simulink model "Copy_of_ENV"  (R2024b)
settings: Solver=FixedStepAuto  StartTime=0.0  StopTime=10.0  RelTol=1e-3  EnableMultiTasking=on
libraries: stm32blockslib x27, canmsglib x9, stm32f4xxblockslib x6, simulink x5
(part 1 of 2)
settings Model: DataDictionary=Master_Dictionary.sldd  STM32="{\"DigitalPortRead\":[{\"ID\":\"ENV:103\"},{\"ID\":\"ENV:734\"}],\"DigitalPortWrite\":[{\"ID\":\"ENV:105\"},{\"ID\":\"ENV:104\"},{\"ID\":\"ENV:735\"},{\"ID\":\"ENV:739\"}],\"SPIControllerTransfer\":[{\"ID\":\"ENV:28\"},{\"ID\":\"ENV:29\"},{\"ID\":\"ENV:30\"},{\"ID\":\"ENV:31\"},{\"ID\":\"ENV:32\"},{\"ID\":\"ENV:33\"},{\"ID\":\"ENV:89\"},{\"ID\":\"ENV:90\"},{\"ID\":\"ENV:91\"},{\"ID\":\"ENV:92\"},{\"ID\":\"ENV:661\"},{\"ID\":\"ENV:662\"},{\"ID\":\"ENV:663\"},{\"ID\":\"ENV:664\"},{\"ID\":\"ENV:665\"},{\"ID\":\"ENV:666\"},{\"ID\":\"ENV:667\"},{\"ID\":\"ENV:668\"},{\"ID\":\"ENV:697\"},{\"ID\":\"ENV:785\"},{\"ID\":\"ENV:784\"},{\"ID\":\"ENV:783\"},{\"ID\":\"ENV:782\"},{\"ID\":\"ENV:781\"},{\"ID\":\"ENV:780\"},{\"ID\":\"ENV:779\"},{\"ID\":\"ENV:778\"}]}"  Creator=Will  LastModifiedBy=Will
settings OptimizationCC: DefaultParameterBehavior=Inlined  EnhancedBackFolding=on  PassReuseOutputArgsAs=Individual arguments  ZeroExternalMemoryAtStartup=off  ZeroInternalMemoryAtStartup=off  MaxStackSize=8192  OptimizeBlockOrder=speed  DifferentSizesBufferReuse=on  OptimizationCustomize=off  EfficientTunableParamExpr=on
settings DebuggingCC: ParameterTunabilityLossMsg=error
settings HardwareCC: ProdBitPerPointer=32  ProdBitPerSizeT=32  ProdBitPerPtrDiffT=32  ProdLargestAtomicInteger=Long  ProdLargestAtomicFloat=Double  ProdWordSize=32  ProdLongLongMode=on  ProdHWDeviceType=ARM Compatible->ARM Cortex-M
settings SFSimCC: MATLABDynamicMemAlloc=off
settings RTWCC: Description=Embedded Coder  SystemTargetFile=ert.tlc  HardwareBoard=STM32H7xx Based (Single-core)  TemplateMakefile=ert_default_tmf  Toolchain=GNU Tools for ARM Embedded Processors
settings CodeAppCC: ForceParamTrailComments=on  IgnoreCustomStorageClasses=off  OperatorAnnotations=on  SimulinkDataObjDesc=on  SFDataObjDesc=on  InsertBlockDesc=on
settings ERTTargetCC: TargetLangStandard=C99 (ISO)  CodeReplacementLibrary=ARM Cortex-M  ExtModeTransport=3  ExtModeStaticAlloc=on  ExtModeStaticAllocSize=2048  ExtModeMexFile=ext_xcp  ExtModeIntrfLevel=Level2 - Open

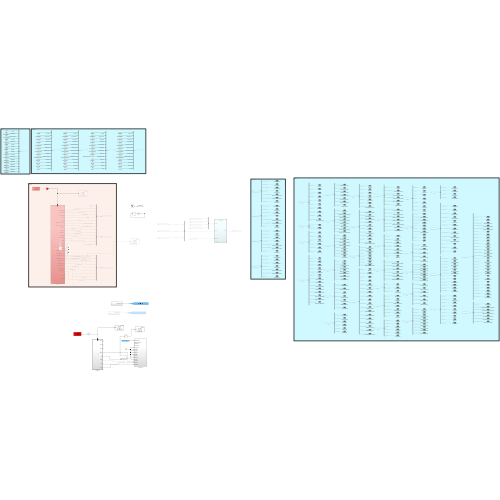
[thumbnail: Simulink's stored preview of the top-level diagram]
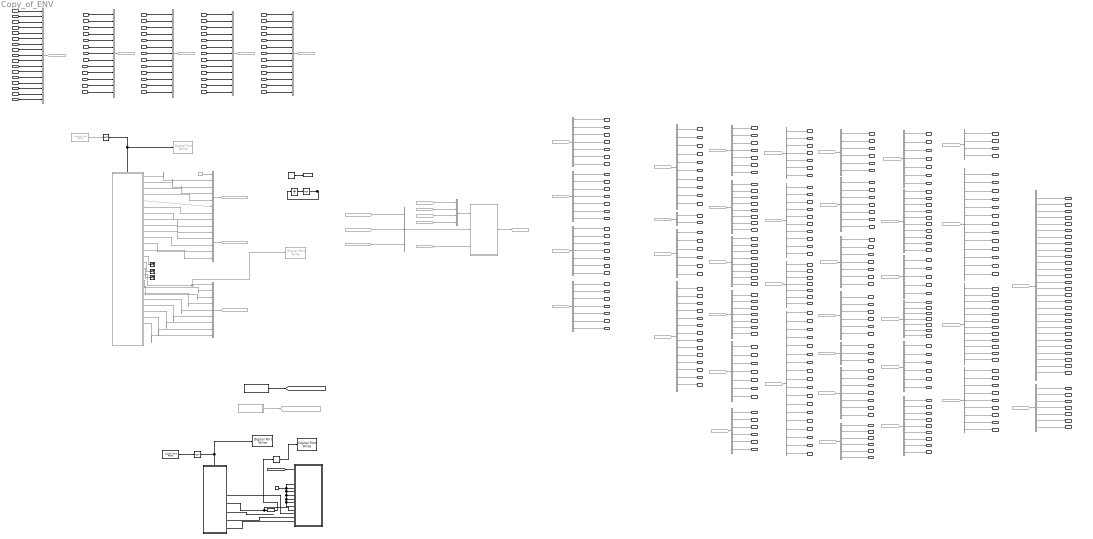
== system Copy_of_ENV ==
  note: CAN3
  note: CAN3
  note: CAN 1&2
  note: CAN1&2
  note: CAN4
  nMotorRL : Inport
  BInvDCOnRLIn : Inport  Port=2
  BInvErrorRL : Inport  Port=3
  BInvOnRLIn : Inport  Port=4
  BInvQuitDcOnRL : Inport  Port=5
  BQuitInvOnRL : Inport  Port=6
  BInvSysReadyRL : Inport  Port=7
  BInvWarnRL : Inport  Port=8
  MMotorMeasuredRL : Inport  Port=9
  NInvDTCRL : Inport  Port=10
  TMotorRL : Inport  Port=11
  VDCInvRL : Inport  Port=12
  TInvRL : Inport  Port=13
  nMotorRR : Inport  Port=14
  BInvDCOnRRIn : Inport  Port=15
  BInvErrorRR : Inport  Port=16
  BInvOnRRIn : Inport  Port=17
  BInvQuitDcOnRR : Inport  Port=18
  BQuitInvOnRR : Inport  Port=19
  BInvSysReadyRR : Inport  Port=20
  BInvWarnRR : Inport  Port=21
  MMotorMeasuredRR : Inport  Port=22
  NInvDTCRR : Inport  Port=23
  TMotorRR : Inport  Port=24
  VDCInvRR : Inport  Port=25
  TInvRR : Inport  Port=26
  nMotorFL : Inport  Port=27
  BInvDCOnFLIn : Inport  Port=28
  BInvErrorFL : Inport  Port=29
  BInvOnFLIn : Inport  Port=30
  BInvQuitDcOnFL : Inport  Port=31
  BQuitInvOnFL : Inport  Port=32
  BInvSysReadyFL : Inport  Port=33
  BInvWarnFL : Inport  Port=34
  MMotorMeasuredFL : Inport  Port=35
  NInvDTCFL : Inport  Port=36
  TMotorFL : Inport  Port=37
  VDCInvFL : Inport  Port=38
  TInvFL : Inport  Port=39
  nMotorFR : Inport  Port=40
  BInvDCOnFRIn : Inport  Port=41
  BInvErrorFR : Inport  Port=42
  BInvOnFRIn : Inport  Port=43
  BInvQuitDcOnFR : Inport  Port=44
  BQuitInvOnFR : Inport  Port=45
  BInvSysReadyFR : Inport  Port=46
  BInvWarnFR : Inport  Port=47
  MMotorMeasuredFR : Inport  Port=48
  NInvDTCFR : Inport  Port=49
  TMotorFR : Inport  Port=50
  VDCInvFR : Inport  Port=51
  TInvFR : Inport  Port=52
  IIVTS : Inport  Port=53
  IBMSHallEffect : Inport  Port=54
  VDCAccumulator : Inport  Port=55
  TCellMin : Inport  Port=56
  VCellAverage : Inport  Port=57
  VCellMax : Inport  Port=58
  TCellMax : Inport  Port=59
  IBMSDCL : Inport  Port=60
  VCellMin : Inport  Port=61
  RCellAverage : Inport  Port=62
  BBalancingOn : Inport  Port=63
  BBMSP0A0C : Inport  Port=64  OutDataTypeStr=boolean
  BBMSP0A0E : Inport  Port=65
  BBMSP0A10 : Inport  Port=66
  BBMSP0A80 : Inport  Port=67
  BBMSP0AC0 : Inport  Port=68
  BBMSP0AFA : Inport  Port=69
  0x1A0 : From  Commented=on  GotoTag=Global
  0x1A1 : From  Commented=on  GotoTag=Global
  0x1A2 : From  Commented=on  GotoTag=Global
  0x{202..203,205..207,210..217,220..223,250..254,300..302,603,700..703} (30 alike) : From  Commented=on  GotoTag=Global
  Bus Creator : BusCreator  Commented=on  Inputs=3  OutDataTypeStr=Bus: CAN3Bus
  Bus Creator14 : BusCreator  Commented=on  Inputs=13  OutDataTypeStr=Bus: InverterFL
  Bus Creator15 : BusCreator  Commented=on  Inputs=13  OutDataTypeStr=Bus: InverterFR
  Bus Creator17 : BusCreator  Commented=on  Inputs=13  OutDataTypeStr=Bus: InverterRL
  Bus Creator18 : BusCreator  Commented=on  Inputs=17  OutDataTypeStr=Bus: BMS
  Bus Creator19 : BusCreator  Commented=on  Inputs=13  OutDataTypeStr=Bus: InverterRR
  Bus Creator2 : BusCreator  Commented=on  Inputs=8  OutDataTypeStr=Bus: DDU7
  Bus Creator3 : BusCreator  Commented=on  Inputs=6  OutDataTypeStr=Bus: IMU
      settings: InheritFromInputs=off
  Bus Creator4 : BusCreator  Commented=on  Inputs=9  OutDataTypeStr=Bus: STW
  Bus Selector : BusSelector  Commented=on  OutputSignals=TorqueControl.MFLFinal,TorqueControl.MFRFinal,TorqueControl.MRLFinal,TorqueControl.MRRFinal,BMSSignals.IIVTS,Systems.PActual,Systems.BBrakeError,Systems.BThrottleError,Systems.BOverpower,Limitations.BDischargeAllowed
  Bus Selector1 : BusSelector  Commented=on  OutputSignals=Systems.vChassis,Systems.PEnergyMeter
  Bus Selector10 : BusSelector  Commented=on  OutputSignals=TorqueControl.MTotalRequested,TorqueControl.rSlipRatioOptimal,TorqueControl.aCamberFL,TorqueControl.aCamberFR,TorqueControl.aCamberRL,TorqueControl.aCamberRR,TorqueControl.FTotalLateralLoadTransfer
  Bus Selector11 : BusSelector  Commented=on  OutputSignals=Systems.BTVOnEM,Systems.BTVOnOW,Systems.BDrivetrainCoolingOn,Systems.BDrivetrainCoolingOnEM,Systems.BDrivetrainCoolingOnOW,Systems.BTCOn,Systems.BTCOnEM,Systems.BTCOnOW,Systems.BEMSOn,Systems.BEMSOnEM,Systems.BEMSOnOW,Systems.BSpinningModeOn,Systems.BSpinningModeOnEM,Systems.BSpinningModeOnOW,Systems.rSOE,BMSSignals.BBalancingOn,BMSSignals.BBMSP0A0C,BMSSignals.BBMSP0A0E,BMSSignals.BBMSP0A10,BMSSignals.BBMSP0A80,BMSSignals.BBMSP0AC0,BMSSignals.BBMSP0AFA,TorqueControl.NLap,Systems.NEventMode,Systems.rTorqueSplit,Systems.NThrottleMap,Systems.NThrottleMapEM,Systems.NThrottleMapOW
  Bus Selector12 : BusSelector  Commented=on  OutputSignals=Systems.aSteeringAngle,Limitations.PLowCellVoltageDischargeDerate,Limitations.PHighCellVoltageRegenDerate,TorqueControl.MDriverDischargeRequested,TorqueControl.MDriverRegenRequested,TorqueControl.PPCIntegralTermDischarge,TorqueControl.PPCIntegralTermRegen
  Bus Selector13 : BusSelector  Commented=on  OutputSignals=Stateflow.NInvState,Systems.BInverterErrorRear,Systems.BInverterErrorFront,Systems.BErrorReset,InverterSignals.InverterRLSignals.TInvRL,InverterSignals.InverterFRSignals.TMotorFR,BMSSignals.VDCAccumulator,TorqueControl.EBudget,TorqueControl.BTVOK,TorqueControl.sSector
  Bus Selector14 : BusSelector  Commented=on  OutputSignals=Systems.sChassis,Limitations.PInvTemperatureDerate,Limitations.PInvTemperatureDerateFR,Limitations.PInvTemperatureDerateFL,Limitations.PInvTemperatureDerateRR,BMSSignals.IBMSHallEffect
  Bus Selector15 : BusSelector  Commented=on  OutputSignals=TorqueControl.NABSMultiplierRR,TorqueControl.MTractionControlRRTotal,TorqueControl.MTotalFinal,TorqueControl.rSlipRatioFLActual,TorqueControl.rSlipRatioFRActual,TorqueControl.rSlipRatioRLActual,TorqueControl.FTyreVerticalFR
  Bus Selector18 : BusSelector  Commented=on  OutputSignals=Systems.PDischargeMax,Systems.PDischargeMaxEM,Systems.PDischargeMaxOW,Systems.PEngineBraking,Systems.PEngineBrakingEM,Systems.PEngineBrakingOW,Systems.rGrip,Systems.EOffset,Systems.NTCKdSelector,Systems.NPCKpSelector,Systems.MRegenMax,Systems.rTorqueSplitEM
  Bus Selector19 : BusSelector  Commented=on  OutputSignals=Systems.tThrottleError,TorqueControl.MTorqueDistributionRR,TorqueControl.NTractionControlMultiplierRL,TorqueControl.NTractionControlMultiplierRR,TorqueControl.NABSMultiplierFL,TorqueControl.NABSMultiplierFR,TorqueControl.NABSMultiplierRL,TorqueControl.FTyreVerticalFL
  Bus Selector2 : BusSelector  Commented=on  OutputSignals=WheelSpeeds.vWheelFL,WheelSpeeds.vWheelFR,InverterSignals.InverterFLSignals.nMotorFL,InverterSignals.InverterFRSignals.nMotorFR,Systems.rThrottlePedal1,Systems.BPageUp,InverterSignals.InverterRLSignals.BQuitInvOnRL,InverterSignals.InverterFLSignals.BQuitInvOnFL,InverterSignals.InverterRRSignals.BQuitInvOnRR,InverterSignals.InverterFRSignals.BQuitInvOnFR,Stateflow.BInvErrorResetRL,Stateflow.BInvErrorResetRR,Stateflow.BInvErrorResetFL,Stateflow.BInvErrorResetFR
  Bus Selector20 : BusSelector  Commented=on  OutputSignals=Stateflow.BInvDCOnRLOut,Stateflow.BInvEnableRL,Stateflow.BInvErrorResetRL,Stateflow.BInvOnRLOut,Stateflow.MTorqueLimitNegativeRL,Stateflow.MTorqueLimitPositiveRL,TorqueControl.MRLFinal
  Bus Selector21 : BusSelector  Commented=on  OutputSignals=Stateflow.BInvDCOnFLOut,Stateflow.BInvEnableFL,Stateflow.BInvErrorResetFL,Stateflow.BInvOnFLOut,Stateflow.MTorqueLimitNegativeFL,Stateflow.MTorqueLimitPositiveFL,TorqueControl.MFLFinal
  Bus Selector22 : BusSelector  Commented=on  OutputSignals=Stateflow.BInvDCOnRROut,Stateflow.BInvEnableRR,Stateflow.BInvErrorResetRR,Stateflow.BInvOnRROut,Stateflow.MTorqueLimitNegativeRR,Stateflow.MTorqueLimitPositiveRR,TorqueControl.MRRFinal
  Bus Selector23 : BusSelector  Commented=on  OutputSignals=Stateflow.BInvDCOnFROut,Stateflow.BInvEnableFR,Stateflow.BInvErrorResetFR,Stateflow.BInvOnFROut,Stateflow.MTorqueLimitNegativeFR,Stateflow.MTorqueLimitPositiveFR,TorqueControl.MFRFinal
  Bus Selector24 : BusSelector  Commented=on  OutputSignals=Systems.tBrakeError,TorqueControl.nYawRateErrorActual,TorqueControl.MTorqueDistributionRL,TorqueControl.MTractionControlRLTotal,TorqueControl.MTractionControlFRTotal,TorqueControl.MTractionControlFLTotal,TorqueControl.rSlipRatioRRActual
  Bus Selector29 : BusSelector  Commented=on  OutputSignals=Stateflow.NCarState,Systems.pBrakeF,Systems.pBrakeR,Systems.tAppsTimer,BMSSignals.VCellMax,BMSSignals.VCellMin,Limitations.PSOCDischargeDerate
  Bus Selector3 : BusSelector  Commented=on  OutputSignals=WheelSpeeds.vWheelRL,WheelSpeeds.vWheelRR,InverterSignals.InverterRLSignals.nMotorRL,InverterSignals.InverterRRSignals.nMotorRR,Systems.rThrottlePedal,Systems.BPageDown
  Bus Selector30 : BusSelector  Commented=on  OutputSignals=Limitations.rSpeedRegenDerateRL,Limitations.rSpeedRegenDerateFR,Limitations.rSpeedRegenDerateFL,Limitations.BSpeedDerateOn,Limitations.PDischargeDerate,Limitations.PRegenDerate,TorqueControl.PRegenRequested,TorqueControl.PDischargeLimit,TorqueControl.PRegenLimit,TorqueControl.PPCDischargeRequested
  Bus Selector31 : BusSelector  Commented=on  OutputSignals=Systems.BPCComplete,Systems.BBrakeLight,Stateflow.BReadyToDriveBuzzer,Systems.BAccuFanOn,Systems.BMotorRBHFanOn,Systems.BInverterFanOn,Systems.BInvLVOn
  Bus Selector33 : BusSelector  Commented=on  OutputSignals=Systems.TMotorMax,Systems.TInvMax,InverterSignals.InverterRLSignals.TMotorRL,InverterSignals.InverterRLSignals.VDCInvRL,InverterSignals.InverterRRSignals.TMotorRR,InverterSignals.InverterFLSignals.TMotorFL
  Bus Selector34 : BusSelector  Commented=on  OutputSignals=TorqueControl.ETotalRequested,TorqueControl.ESector1Remaining,TorqueControl.ESector2Remaining,TorqueControl.ESector3Remaining,TorqueControl.ESector4Remaining
  Bus Selector35 : BusSelector  Commented=on  OutputSignals=TorqueControl.ERemaining,TorqueControl.FTotalDownforce,TorqueControl.aCamberGainRollF,TorqueControl.aCamberGainRollR,TorqueControl.aCamberGainHeaveF,TorqueControl.aCamberGainHeaveR,TorqueControl.aRollAngle
  Bus Selector38 : BusSelector  Commented=on  OutputSignals=TorqueControl.NSectorGlobal,TorqueControl.NSectorLap,TorqueControl.NSector3Remaining,TorqueControl.NSector4Remaining,TorqueControl.NSector5Remaining,TorqueControl.NSector6Remaining,TorqueControl.NSector7Remaining,TorqueControl.NSector8Remaining,TorqueControl.ESector8Remaining
  Bus Selector4 : BusSelector  Commented=on  OutputSignals=Systems.tPedalOverlap,TorqueControl.PPCProportionalTermDischarge,TorqueControl.MPCDischargeRequested,TorqueControl.PPCProportionalTermRegen,TorqueControl.MPCRegenRequested,TorqueControl.MDischargeLimited,TorqueControl.NTractionControlMultiplierFL,TorqueControl.NTractionControlMultiplierFR
  Bus Selector42 : BusSelector  Commented=on  OutputSignals=Limitations.PInvTemperatureDerateRL,Limitations.PMotorTemperatureDerate,Limitations.PMotorTemperatureDerateFR,Limitations.PMotorTemperatureDerateFL,Limitations.PMotorTemperatureDerateRR,TorqueControl.aCamberGainSteerFL,TorqueControl.aCamberGainSteerFR
  Bus Selector47 : BusSelector  Commented=on  OutputSignals=Limitations.PMotorTemperatureDerateRL,Limitations.PTSTemperatureDerateFR,Limitations.PTSTemperatureDerateFL,Limitations.PTSTemperatureDerateRR,Limitations.PTSTemperatureDerateRL,Limitations.PHighCellTemperatureDerate
  Bus Selector48 : BusSelector  Commented=on  OutputSignals=TorqueControl.ESector,TorqueControl.xHeaveTravelF,TorqueControl.xHeaveTravelR
  Bus Selector49 : BusSelector  Commented=on  OutputSignals=Stateflow.NBMSState,InverterSignals.InverterRRSignals.TInvRR,InverterSignals.InverterFLSignals.TInvFL,InverterSignals.InverterFRSignals.TInvFR,BMSSignals.TCellMax,BMSSignals.TCellMin,TorqueControl.rSplitRear
  Bus Selector5 : BusSelector  Commented=on  OutputSignals=Systems.pBrakeMax,Systems.rRegenPaddle,Systems.xDamperFL,Systems.xDamperFR,Systems.xDamperRL,Systems.xDamperRR,Systems.BIMUOK,Systems.tIMUError,Systems.BDataMark
  Bus Selector53 : BusSelector  Commented=on  OutputSignals=TorqueControl.ESector9Remaining,TorqueControl.ESector10Remaining,TorqueControl.ESector11Remaining,TorqueControl.ESector12Remaining,TorqueControl.NSector1Remaining,TorqueControl.NSector2Remaining
  Bus Selector54 : BusSelector  Commented=on  OutputSignals=TorqueControl.NSector9Remaining,TorqueControl.NSector10Remaining,TorqueControl.NSector11Remaining,TorqueControl.NSector12Remaining,TorqueControl.ESector5Remaining,TorqueControl.ESector6Remaining,TorqueControl.ESector7Remaining
  Bus Selector55 : BusSelector  Commented=on  OutputSignals=Systems.rTorqueSplitOW,Systems.PRegenMax,Systems.PRegenMaxEM,Systems.PRegenMaxOW,Systems.rTVMultiplier,Systems.rTVMultiplierEM,Systems.rTVMultiplierOW,Systems.rEngineBrakingSplit,Systems.rEngineBrakingSplitEM,Systems.rEngineBrakingSplitOW,Systems.rSOC,Stateflow.BReadyToDrive,Systems.BTVOn
  Bus Selector6 : BusSelector  Commented=on  OutputSignals=TorqueControl.FTyreVerticalRL,TorqueControl.FTyreVerticalRR,TorqueControl.aSlipAngleFL,TorqueControl.aSlipAngleFR,TorqueControl.aSlipAngleRL,TorqueControl.aSlipAngleRR
  Bus Selector7 : BusSelector  Commented=on  OutputSignals=InverterSignals.InverterRLSignals.NInvDTCRL,InverterSignals.InverterRRSignals.NInvDTCRR,InverterSignals.InverterFLSignals.NInvDTCFL,InverterSignals.InverterFRSignals.NInvDTCFR
  Bus Selector8 : BusSelector  Commented=on  OutputSignals=Systems.BBrakeOn,Systems.BPedalOverlap,Systems.BAppsOK,Systems.BRegenOn,Systems.BxDamperFLOk,Systems.BxDamperFROk,Systems.BxDamperRLOk,Systems.BxDamperRROk,Systems.BIMUError,Systems.BCalibrationOn,Limitations.PSOCRegenDerate,Limitations.rSpeedRegenDerateRR,TorqueControl.PPCRegenRequested,TorqueControl.PDischargeLimited,TorqueControl.BEMSDriverSignal1,TorqueControl.BEMSDriverSignal2,TorqueControl.BEMSDriverSignal3,TorqueControl.FLongitudinalLoadTransfer
  Bus Selector9 : BusSelector  Commented=on  OutputSignals=TorqueControl.MTorqueVectoringFL,TorqueControl.MTorqueVectoringFR,TorqueControl.MTorqueVectoringRL,TorqueControl.MTorqueVectoringRR,TorqueControl.MTorqueDistributionFL,TorqueControl.MTorqueDistributionFR,TorqueControl.MRegenLimited
  CAN Rx : Subsystem  Commented=on  TreatAsAtomicUnit=on
  CAN Rx1 : Subsystem  TreatAsAtomicUnit=on
  CAN Tx20 : Subsystem
  CAN1_2Bus : BusCreator  Commented=on  Inputs=4  OutDataTypeStr=Bus: CAN1_2Bus
  Compare To Constant : simulink/Logic and Bit Operations/Compare To Constant  relop=>=  const=125  OutDataTypeStr=boolean
  Compare To Constant1 : simulink/Logic and Bit Operations/Compare To Constant  relop===  const=5  OutDataTypeStr=boolean
  Constant2 : Constant  Commented=on  Value=69
  Constant3 : Constant  Value=0
  Counter Limited : simulink/Sources/Counter Limited  uplimit=250  tsamp=-1
  Data Type Conversion : DataTypeConversion  OutDataTypeStr=double  SaturateOnIntegerOverflow=off  RndMeth=Floor
  Digital Port Read1 : stm32f4xxblockslib/Digital Port Read  Commented=on  PortName=GPIOA  PinNumber=2  ReadOperation=on  IOAsArray=off  SampleTime=-1  EnableSimPort=off  hoistedMaskSrc=ECSoC/ECSimCodegen/Digital Port Read
      settings: LibrarySourceBlock=stm32f2xxblockslib/Digital Port Read
  Digital Port Read3 : stm32f4xxblockslib/Digital Port Read  PortName=GPIOA  PinNumber=2  ReadOperation=on  IOAsArray=off  SampleTime=-1  EnableSimPort=off  hoistedMaskSrc=ECSoC/ECSimCodegen/Digital Port Read
      settings: LibrarySourceBlock=stm32f2xxblockslib/Digital Port Read
  Digital Port Write : stm32f4xxblockslib/Digital Port Write  Commented=on  PortName=GPIOB  PinNumber=4  ReadOperation=off  IOAsArray=off  EnableSimPort=off  hoistedMaskSrc=ECSoC/ECSimCodegen/Digital Port Write
      settings: LibrarySourceBlock=stm32h7xxblockslib/Digital Port Write
  Digital Port Write1 : stm32f4xxblockslib/Digital Port Write  Commented=on  PortName=GPIOB  PinNumber=5  ReadOperation=off  IOAsArray=off  EnableSimPort=off  hoistedMaskSrc=ECSoC/ECSimCodegen/Digital Port Write
      settings: LibrarySourceBlock=stm32h7xxblockslib/Digital Port Write
  Digital Port Write2 : stm32f4xxblockslib/Digital Port Write  PortName=GPIOB  PinNumber=4  ReadOperation=off  IOAsArray=off  EnableSimPort=off  hoistedMaskSrc=ECSoC/ECSimCodegen/Digital Port Write
      settings: LibrarySourceBlock=stm32h7xxblockslib/Digital Port Write
  Digital Port Write3 : stm32f4xxblockslib/Digital Port Write  PortName=GPIOB  PinNumber=5  ReadOperation=off  IOAsArray=off  EnableSimPort=off  hoistedMaskSrc=ECSoC/ECSimCodegen/Digital Port Write
      settings: LibrarySourceBlock=stm32h7xxblockslib/Digital Port Write
  From : From  Commented=on  GotoTag=BMS
  From1 : From  Commented=on  GotoTag=InverterFL
  From2 : From  Commented=on  GotoTag=InverterFR
  From3 : From  Commented=on  GotoTag=InverterRR
  From4 : From  Commented=on  GotoTag=InverterRL
  From5 : From  Commented=on  GotoTag=DDU7
  From6 : From  Commented=on  GotoTag=STW
  From7 : From  Commented=on  GotoTag=IMU
  Goto : Goto  Commented=on  GotoTag=InverterRL
  Goto1 : Goto  Commented=on  GotoTag=InverterRR
  Goto17 : Goto  Commented=on  GotoTag=Global
  Goto2 : Goto  Commented=on  GotoTag=InverterFL
  Goto21 : Goto  Commented=on  GotoTag=MCPInitialized
  Goto3 : Goto  Commented=on  GotoTag=InverterFR
  Goto4 : Goto  Commented=on  GotoTag=BMS
  Goto6 : Goto  Commented=on  GotoTag=DDU7
  Goto8 : Goto  Commented=on  GotoTag=IMU
  Goto9 : Goto  Commented=on  GotoTag=STW
  INV1_Recieve_1 : From  Commented=on  GotoTag=Global
  INV2_Recieve_1 : From  Commented=on  GotoTag=Global
  INV3_Recieve_1 : From  Commented=on  GotoTag=Global
  INV4_Recieve_1 : From  Commented=on  GotoTag=Global
  Model : ModelReference  Commented=on  ModelNameDialog=MASTER.slx  SimulationMode=Normal  ModelReferenceVersion=13.12
  NOT : Logic  Operator=NOT  IconShape=distinctive  AllPortsSameDT=off  OutDataTypeStr=boolean
  NOT1 : Logic  Operator=NOT  IconShape=distinctive  AllPortsSameDT=off  OutDataTypeStr=boolean
  NOT4 : Logic  Operator=NOT  IconShape=distinctive  AllPortsSameDT=off  OutDataTypeStr=boolean
  Subsystem : Subsystem  Commented=on
  Subsystem1 : Subsystem
  Terminator : Terminator
  Terminator1 : Terminator
  Terminator2 : Terminator
  Unit Delay : UnitDelay  SampleTime=-1  HasFrameUpgradeWarning=on
  MTotalFinal : Outport  VectorParamsAs1DForOutWhenUnconnected=off
  PActual : Outport  Port=2  VectorParamsAs1DForOutWhenUnconnected=off
  rSpeedRegenDerateRR : Outport  Port=3  VectorParamsAs1DForOutWhenUnconnected=off
  PDischargeMax : Outport  Port=4  VectorParamsAs1DForOutWhenUnconnected=off
  rThrottlePedal : Outport  Port=5  VectorParamsAs1DForOutWhenUnconnected=off
  rThrottlePedal1 : Outport  Port=6  VectorParamsAs1DForOutWhenUnconnected=off
  aSteeringAngle : Outport  Port=7  VectorParamsAs1DForOutWhenUnconnected=off
  pBrakeF : Outport  Port=8  VectorParamsAs1DForOutWhenUnconnected=off
  pBrakeR : Outport  Port=9  VectorParamsAs1DForOutWhenUnconnected=off
  BBMSP0A80Out : Outport  Port=10  VectorParamsAs1DForOutWhenUnconnected=off
  BBMSP0AC0Out : Outport  Port=11  VectorParamsAs1DForOutWhenUnconnected=off
  BBMSP0AFAOut : Outport  Port=12  VectorParamsAs1DForOutWhenUnconnected=off
  BBMSP0A0COut : Outport  Port=13  VectorParamsAs1DForOutWhenUnconnected=off
  BBMSP0A0EOut : Outport  Port=14  VectorParamsAs1DForOutWhenUnconnected=off
  BBMSP0A10Out : Outport  Port=15  VectorParamsAs1DForOutWhenUnconnected=off
  BTVOK : Outport  Port=16  VectorParamsAs1DForOutWhenUnconnected=off
  NInvDTCRROut : Outport  Port=17  VectorParamsAs1DForOutWhenUnconnected=off
  NInvDTCRLOut : Outport  Port=18  VectorParamsAs1DForOutWhenUnconnected=off
  NInvDTCFROut : Outport  Port=19  VectorParamsAs1DForOutWhenUnconnected=off
  NInvDTCFLOut : Outport  Port=20  VectorParamsAs1DForOutWhenUnconnected=off
  IIVTSOut : Outport  Port=21  VectorParamsAs1DForOutWhenUnconnected=off
  MFRFinal : Outport  Port=22  VectorParamsAs1DForOutWhenUnconnected=off
  MFLFinal : Outport  Port=23  VectorParamsAs1DForOutWhenUnconnected=off
  MRLFinal : Outport  Port=24  VectorParamsAs1DForOutWhenUnconnected=off
  MRRFinal : Outport  Port=25  VectorParamsAs1DForOutWhenUnconnected=off
  rRegenPaddle : Outport  Port=26  VectorParamsAs1DForOutWhenUnconnected=off
  vChassis : Outport  Port=27  VectorParamsAs1DForOutWhenUnconnected=off
  pBrakeMax : Outport  Port=28  VectorParamsAs1DForOutWhenUnconnected=off
  vWheelRL : Outport  Port=29  VectorParamsAs1DForOutWhenUnconnected=off
  vWheelRR : Outport  Port=30  VectorParamsAs1DForOutWhenUnconnected=off
  vWheelFL : Outport  Port=31  VectorParamsAs1DForOutWhenUnconnected=off
  vWheelFR : Outport  Port=32  VectorParamsAs1DForOutWhenUnconnected=off
  BThrottleError : Outport  Port=33  VectorParamsAs1DForOutWhenUnconnected=off
  tThrottleError : Outport  Port=34  VectorParamsAs1DForOutWhenUnconnected=off
  BBrakeError : Outport  Port=35  VectorParamsAs1DForOutWhenUnconnected=off
  tBrakeError : Outport  Port=36  VectorParamsAs1DForOutWhenUnconnected=off
  BBrakeOn : Outport  Port=37  VectorParamsAs1DForOutWhenUnconnected=off
  BPedalOverlap : Outport  Port=38  VectorParamsAs1DForOutWhenUnconnected=off
  BAppsOK : Outport  Port=39  VectorParamsAs1DForOutWhenUnconnected=off
  BRegenOn : Outport  Port=40  VectorParamsAs1DForOutWhenUnconnected=off
  BTVOn : Outport  Port=41  VectorParamsAs1DForOutWhenUnconnected=off
  rSOE : Outport  Port=42  VectorParamsAs1DForOutWhenUnconnected=off
  sChassis : Outport  Port=43  VectorParamsAs1DForOutWhenUnconnected=off
  rSOC : Outport  Port=44  VectorParamsAs1DForOutWhenUnconnected=off
  rTVMultiplier : Outport  Port=45  VectorParamsAs1DForOutWhenUnconnected=off
  PEngineBraking : Outport  Port=46  VectorParamsAs1DForOutWhenUnconnected=off
  NInvState : Outport  Port=47  VectorParamsAs1DForOutWhenUnconnected=off
  rGrip : Outport  Port=48  VectorParamsAs1DForOutWhenUnconnected=off
  rSlipRatioFRActual : Outport  Port=49  VectorParamsAs1DForOutWhenUnconnected=off
  rSlipRatioRLActual : Outport  Port=50  VectorParamsAs1DForOutWhenUnconnected=off
  rSlipRatioRRActual : Outport  Port=51  VectorParamsAs1DForOutWhenUnconnected=off
  NTractionControlMultiplierRR : Outport  Port=52  VectorParamsAs1DForOutWhenUnconnected=off
  NABSMultiplierRR : Outport  Port=53  VectorParamsAs1DForOutWhenUnconnected=off
  NTractionControlMultiplierRL : Outport  Port=54  VectorParamsAs1DForOutWhenUnconnected=off
  NABSMultiplierRL : Outport  Port=55  VectorParamsAs1DForOutWhenUnconnected=off
  NThrottleMap : Outport  Port=56  VectorParamsAs1DForOutWhenUnconnected=off
  BReadyToDrive : Outport  Port=57  VectorParamsAs1DForOutWhenUnconnected=off
  NABSMultiplierFL : Outport  Port=58  VectorParamsAs1DForOutWhenUnconnected=off
  NABSMultiplierFR : Outport  Port=59  VectorParamsAs1DForOutWhenUnconnected=off
  BBalancingOnOut : Outport  Port=60  VectorParamsAs1DForOutWhenUnconnected=off
  MTorqueVectoringFL : Outport  Port=61  VectorParamsAs1DForOutWhenUnconnected=off
  MTorqueVectoringFR : Outport  Port=62  VectorParamsAs1DForOutWhenUnconnected=off
  MTorqueVectoringRL : Outport  Port=63  VectorParamsAs1DForOutWhenUnconnected=off
  MTorqueVectoringRR : Outport  Port=64  VectorParamsAs1DForOutWhenUnconnected=off
  NTractionControlMultiplierFL : Outport  Port=65  VectorParamsAs1DForOutWhenUnconnected=off
  NTractionControlMultiplierFR : Outport  Port=66  VectorParamsAs1DForOutWhenUnconnected=off
  MDischargeLimited : Outport  Port=67  VectorParamsAs1DForOutWhenUnconnected=off
  MDriverRegenRequested : Outport  Port=68  VectorParamsAs1DForOutWhenUnconnected=off
  rSlipRatioOptimal : Outport  Port=69  VectorParamsAs1DForOutWhenUnconnected=off
  NCarState : Outport  Port=70  VectorParamsAs1DForOutWhenUnconnected=off
  MTorqueDistributionFL : Outport  Port=71  VectorParamsAs1DForOutWhenUnconnected=off
  MTorqueDistributionFR : Outport  Port=72  VectorParamsAs1DForOutWhenUnconnected=off
  MTorqueDistributionRL : Outport  Port=73  VectorParamsAs1DForOutWhenUnconnected=off
  MTorqueDistributionRR : Outport  Port=74  VectorParamsAs1DForOutWhenUnconnected=off
  nMotorRLOut : Outport  Port=75  VectorParamsAs1DForOutWhenUnconnected=off
  nMotorFLOut : Outport  Port=76  VectorParamsAs1DForOutWhenUnconnected=off
  nMotorRROut : Outport  Port=77  VectorParamsAs1DForOutWhenUnconnected=off
  nMotorFROut : Outport  Port=78  VectorParamsAs1DForOutWhenUnconnected=off
  BDischargeAllowed : Outport  Port=79  VectorParamsAs1DForOutWhenUnconnected=off
  TMotorRLOut : Outport  Port=80  VectorParamsAs1DForOutWhenUnconnected=off
  TInvRLOut : Outport  Port=81  VectorParamsAs1DForOutWhenUnconnected=off
  TMotorFLOut : Outport  Port=82  VectorParamsAs1DForOutWhenUnconnected=off
  TInvFLOut : Outport  Port=83  VectorParamsAs1DForOutWhenUnconnected=off
  TMotorRROut : Outport  Port=84  VectorParamsAs1DForOutWhenUnconnected=off
  TInvRROut : Outport  Port=85  VectorParamsAs1DForOutWhenUnconnected=off
  TMotorFROut : Outport  Port=86  VectorParamsAs1DForOutWhenUnconnected=off
  TInvFROut : Outport  Port=87  VectorParamsAs1DForOutWhenUnconnected=off
  TInvMax : Outport  Port=88  VectorParamsAs1DForOutWhenUnconnected=off
  TMotorMax : Outport  Port=89  VectorParamsAs1DForOutWhenUnconnected=off
  TCellMaxOut : Outport  Port=90  VectorParamsAs1DForOutWhenUnconnected=off
  IBMSHallEffectOut : Outport  Port=91  VectorParamsAs1DForOutWhenUnconnected=off
  VDCInvRLOut : Outport  Port=92  VectorParamsAs1DForOutWhenUnconnected=off
  BEMSOn : Outport  Port=93  VectorParamsAs1DForOutWhenUnconnected=off
  BTCOn : Outport  Port=94  VectorParamsAs1DForOutWhenUnconnected=off
  VCellMinOut : Outport  Port=95  VectorParamsAs1DForOutWhenUnconnected=off
  VCellMaxOut : Outport  Port=96  VectorParamsAs1DForOutWhenUnconnected=off
  TCellMinOut : Outport  Port=97  VectorParamsAs1DForOutWhenUnconnected=off
  nYawRateErrorActual : Outport  Port=98  VectorParamsAs1DForOutWhenUnconnected=off
  tPedalOverlap : Outport  Port=99  VectorParamsAs1DForOutWhenUnconnected=off
  tAppsTimer : Outport  Port=100  VectorParamsAs1DForOutWhenUnconnected=off
  rSplitRear : Outport  Port=101  VectorParamsAs1DForOutWhenUnconnected=off
  PRegenLimit : Outport  Port=102  VectorParamsAs1DForOutWhenUnconnected=off
  PRegenRequested : Outport  Port=103  VectorParamsAs1DForOutWhenUnconnected=off
  BIMUOk : Outport  Port=104  VectorParamsAs1DForOutWhenUnconnected=off
  EOffset : Outport  Port=105  VectorParamsAs1DForOutWhenUnconnected=off
  PEnergyMeter : Outport  Port=106  VectorParamsAs1DForOutWhenUnconnected=off
  NBMSState : Outport  Port=107  VectorParamsAs1DForOutWhenUnconnected=off
  BOverpower : Outport  Port=108  VectorParamsAs1DForOutWhenUnconnected=off
  BPCComplete : Outport  Port=109  VectorParamsAs1DForOutWhenUnconnected=off
  BEMSDriverSignal1 : Outport  Port=110  VectorParamsAs1DForOutWhenUnconnected=off
  BEMSDriverSignal2 : Outport  Port=111  VectorParamsAs1DForOutWhenUnconnected=off
  BEMSDriverSignal3 : Outport  Port=112  VectorParamsAs1DForOutWhenUnconnected=off
  BPageUp : Outport  Port=113  VectorParamsAs1DForOutWhenUnconnected=off
  BPageDown : Outport  Port=114  VectorParamsAs1DForOutWhenUnconnected=off
  MRegenMax : Outport  Port=115  VectorParamsAs1DForOutWhenUnconnected=off
  NSectorLap : Outport  Port=116  VectorParamsAs1DForOutWhenUnconnected=off
  MPCRegenRequested : Outport  Port=117  VectorParamsAs1DForOutWhenUnconnected=off
  MPCDischargeRequested : Outport  Port=118  VectorParamsAs1DForOutWhenUnconnected=off
  PPCIntegralTermDischarge : Outport  Port=119  VectorParamsAs1DForOutWhenUnconnected=off
  PPCIntegralTermRegen : Outport  Port=120  VectorParamsAs1DForOutWhenUnconnected=off
  NSectorGlobal : Outport  Port=121  VectorParamsAs1DForOutWhenUnconnected=off
  PPCProportionalTermDischarge : Outport  Port=122  VectorParamsAs1DForOutWhenUnconnected=off
  PPCProportionalTermRegen : Outport  Port=123  VectorParamsAs1DForOutWhenUnconnected=off
  BDataMark : Outport  Port=124  VectorParamsAs1DForOutWhenUnconnected=off
  xDamperFL : Outport  Port=125  VectorParamsAs1DForOutWhenUnconnected=off
  xDamperFR : Outport  Port=126  VectorParamsAs1DForOutWhenUnconnected=off
  xDamperRR : Outport  Port=127  VectorParamsAs1DForOutWhenUnconnected=off
  xDamperRL : Outport  Port=128  VectorParamsAs1DForOutWhenUnconnected=off
  BErrorReset : Outport  Port=129  VectorParamsAs1DForOutWhenUnconnected=off
  BDrivetrainCoolingOn : Outport  Port=130  VectorParamsAs1DForOutWhenUnconnected=off
  PPCRegenRequested : Outport  Port=131  VectorParamsAs1DForOutWhenUnconnected=off
  PDischargeLimit : Outport  Port=132  VectorParamsAs1DForOutWhenUnconnected=off
  PRegenDerate : Outport  Port=133  VectorParamsAs1DForOutWhenUnconnected=off
  PHighCellVoltageRegenDerate : Outport  Port=134  VectorParamsAs1DForOutWhenUnconnected=off
  PHighCellTemperatureDerate : Outport  Port=135  VectorParamsAs1DForOutWhenUnconnected=off
  PDischargeDerate : Outport  Port=136  VectorParamsAs1DForOutWhenUnconnected=off
  PMotorTemperatureDerate : Outport  Port=137  VectorParamsAs1DForOutWhenUnconnected=off
  PMotorTemperatureDerateFL : Outport  Port=138  VectorParamsAs1DForOutWhenUnconnected=off
  PMotorTemperatureDerateFR : Outport  Port=139  VectorParamsAs1DForOutWhenUnconnected=off
  PMotorTemperatureDerateRL : Outport  Port=140  VectorParamsAs1DForOutWhenUnconnected=off
  PMotorTemperatureDerateRR : Outport  Port=141  VectorParamsAs1DForOutWhenUnconnected=off
  PLowCellVoltageDischargeDerate : Outport  Port=142  VectorParamsAs1DForOutWhenUnconnected=off
  PInvTemperatureDerate : Outport  Port=143  VectorParamsAs1DForOutWhenUnconnected=off
  PInvTemperatureDerateFL : Outport  Port=144  VectorParamsAs1DForOutWhenUnconnected=off
  PInvTemperatureDerateFR : Outport  Port=145  VectorParamsAs1DForOutWhenUnconnected=off
  PInvTemperatureDerateRR : Outport  Port=146  VectorParamsAs1DForOutWhenUnconnected=off
  PInvTemperatureDerateRL : Outport  Port=147  VectorParamsAs1DForOutWhenUnconnected=off
  aCamberGainSteerFL : Outport  Port=148  VectorParamsAs1DForOutWhenUnconnected=off
  aCamberGainSteerFR : Outport  Port=149  VectorParamsAs1DForOutWhenUnconnected=off
  PPCDischargeRequested : Outport  Port=150  VectorParamsAs1DForOutWhenUnconnected=off
  rSlipRatioFLActual : Outport  Port=151  VectorParamsAs1DForOutWhenUnconnected=off
  FLongitudinalLoadTransfer : Outport  Port=152  VectorParamsAs1DForOutWhenUnconnected=off
  FTyreVerticalFL : Outport  Port=153  VectorParamsAs1DForOutWhenUnconnected=off
  FTyreVerticalFR : Outport  Port=154  VectorParamsAs1DForOutWhenUnconnected=off
  FTyreVerticalRL : Outport  Port=155  VectorParamsAs1DForOutWhenUnconnected=off
  FTyreVerticalRR : Outport  Port=156  VectorParamsAs1DForOutWhenUnconnected=off
  BCalibrationOn : Outport  Port=157  VectorParamsAs1DForOutWhenUnconnected=off
  FTotalDownforce : Outport  Port=158  VectorParamsAs1DForOutWhenUnconnected=off
  aSlipAngleFL : Outport  Port=159  VectorParamsAs1DForOutWhenUnconnected=off
  aSlipAngleFR : Outport  Port=160  VectorParamsAs1DForOutWhenUnconnected=off
  aCamberFL : Outport  Port=161  VectorParamsAs1DForOutWhenUnconnected=off
  aCamberFR : Outport  Port=162  VectorParamsAs1DForOutWhenUnconnected=off
  aCamberRL : Outport  Port=163  VectorParamsAs1DForOutWhenUnconnected=off
  aCamberRR : Outport  Port=164  VectorParamsAs1DForOutWhenUnconnected=off
  aRollAngle : Outport  Port=165  VectorParamsAs1DForOutWhenUnconnected=off
  xHeaveTravelR : Outport  Port=166  VectorParamsAs1DForOutWhenUnconnected=off
  xHeaveTravelF : Outport  Port=167  VectorParamsAs1DForOutWhenUnconnected=off
  rSpeedRegenDerateFR : Outport  Port=168  VectorParamsAs1DForOutWhenUnconnected=off
  rSpeedRegenDerateRL : Outport  Port=169  VectorParamsAs1DForOutWhenUnconnected=off
  rSpeedRegenDerateFL : Outport  Port=170  VectorParamsAs1DForOutWhenUnconnected=off
  PTSTemperatureDerateFL : Outport  Port=171  VectorParamsAs1DForOutWhenUnconnected=off
  PTSTemperatureDerateFR : Outport  Port=172  VectorParamsAs1DForOutWhenUnconnected=off
  PTSTemperatureDerateRL : Outport  Port=173  VectorParamsAs1DForOutWhenUnconnected=off
  PTSTemperatureDerateRR : Outport  Port=174  VectorParamsAs1DForOutWhenUnconnected=off
  PSOCDischargeDerate : Outport  Port=175  VectorParamsAs1DForOutWhenUnconnected=off
  PSOCRegenDerate : Outport  Port=176  VectorParamsAs1DForOutWhenUnconnected=off
  aSlipAngleRL : Outport  Port=177  VectorParamsAs1DForOutWhenUnconnected=off
  aSlipAngleRR : Outport  Port=178  VectorParamsAs1DForOutWhenUnconnected=off
  BSpeedDerateOn : Outport  Port=179  VectorParamsAs1DForOutWhenUnconnected=off
  VDCAccumulatorOut : Outport  Port=180  VectorParamsAs1DForOutWhenUnconnected=off
  MTractionControlRRTotal : Outport  Port=181  VectorParamsAs1DForOutWhenUnconnected=off
  MTractionControlRLTotal : Outport  Port=182  VectorParamsAs1DForOutWhenUnconnected=off
  MTractionControlFRTotal : Outport  Port=183  VectorParamsAs1DForOutWhenUnconnected=off
  MTractionControlFLTotal : Outport  Port=184  VectorParamsAs1DForOutWhenUnconnected=off
  BSpinningModeOn : Outport  Port=185  VectorParamsAs1DForOutWhenUnconnected=off
  PRegenMax : Outport  Port=186  VectorParamsAs1DForOutWhenUnconnected=off
  rEngineBrakingSplit : Outport  Port=187  VectorParamsAs1DForOutWhenUnconnected=off
  NLap : Outport  Port=188  VectorParamsAs1DForOutWhenUnconnected=off
  sSector : Outport  Port=189  VectorParamsAs1DForOutWhenUnconnected=off
  EBudget : Outport  Port=190  VectorParamsAs1DForOutWhenUnconnected=off
  ERemaining : Outport  Port=191  VectorParamsAs1DForOutWhenUnconnected=off
  ESector : Outport  Port=192  VectorParamsAs1DForOutWhenUnconnected=off
  FTotalLateralLoadTransfer : Outport  Port=193  VectorParamsAs1DForOutWhenUnconnected=off
  BAccuFanOn : Outport  Port=194  VectorParamsAs1DForOutWhenUnconnected=off
  BMotorRBHFanOn : Outport  Port=195  VectorParamsAs1DForOutWhenUnconnected=off
  BInverterFanOn : Outport  Port=196  VectorParamsAs1DForOutWhenUnconnected=off
  BReadyToDriveBuzzer : Outport  Port=197  VectorParamsAs1DForOutWhenUnconnected=off
  BBrakeLight : Outport  Port=198  VectorParamsAs1DForOutWhenUnconnected=off
  BInvLVOn : Outport  Port=199  VectorParamsAs1DForOutWhenUnconnected=off
  tIMUError : Outport  Port=200  VectorParamsAs1DForOutWhenUnconnected=off
  MDriverDischargeRequested : Outport  Port=201  VectorParamsAs1DForOutWhenUnconnected=off
  MRegenLimited : Outport  Port=202  VectorParamsAs1DForOutWhenUnconnected=off
  MTotalRequested : Outport  Port=203  VectorParamsAs1DForOutWhenUnconnected=off
  BxDamperFLOk : Outport  Port=204  VectorParamsAs1DForOutWhenUnconnected=off
  BxDamperFROk : Outport  Port=205  VectorParamsAs1DForOutWhenUnconnected=off
  BxDamperRLOk : Outport  Port=206  VectorParamsAs1DForOutWhenUnconnected=off
  BxDamperRROk : Outport  Port=207  VectorParamsAs1DForOutWhenUnconnected=off
  BIMUError : Outport  Port=208  VectorParamsAs1DForOutWhenUnconnected=off
  PDischargeLimited : Outport  Port=209  VectorParamsAs1DForOutWhenUnconnected=off
  aCamberGainRollF : Outport  Port=210  VectorParamsAs1DForOutWhenUnconnected=off
  aCamberGainRollR : Outport  Port=211  VectorParamsAs1DForOutWhenUnconnected=off
  aCamberGainHeaveF : Outport  Port=212  VectorParamsAs1DForOutWhenUnconnected=off
  aCamberGainHeaveR : Outport  Port=213  VectorParamsAs1DForOutWhenUnconnected=off
  BInverterErrorRear : Outport  Port=214  VectorParamsAs1DForOutWhenUnconnected=off
  BInverterErrorFront : Outport  Port=215  VectorParamsAs1DForOutWhenUnconnected=off
  ETotalRequested : Outport  Port=216  VectorParamsAs1DForOutWhenUnconnected=off
  ESector1Remaining : Outport  Port=217  VectorParamsAs1DForOutWhenUnconnected=off
  ESector2Remaining : Outport  Port=218  VectorParamsAs1DForOutWhenUnconnected=off
  ESector3Remaining : Outport  Port=219  VectorParamsAs1DForOutWhenUnconnected=off
  ESector4Remaining : Outport  Port=220  VectorParamsAs1DForOutWhenUnconnected=off
  NSector9Remaining : Outport  Port=221  VectorParamsAs1DForOutWhenUnconnected=off
  NSector10Remaining : Outport  Port=222  VectorParamsAs1DForOutWhenUnconnected=off
  NSector11Remaining : Outport  Port=223  VectorParamsAs1DForOutWhenUnconnected=off
  NSector12Remaining : Outport  Port=224  VectorParamsAs1DForOutWhenUnconnected=off
  ESector5Remaining : Outport  Port=225  VectorParamsAs1DForOutWhenUnconnected=off
  ESector6Remaining : Outport  Port=226  VectorParamsAs1DForOutWhenUnconnected=off
  ESector7Remaining : Outport  Port=227  VectorParamsAs1DForOutWhenUnconnected=off
  ESector9Remaining : Outport  Port=228  VectorParamsAs1DForOutWhenUnconnected=off
  ESector10Remaining : Outport  Port=229  VectorParamsAs1DForOutWhenUnconnected=off
  ESector11Remaining : Outport  Port=230  VectorParamsAs1DForOutWhenUnconnected=off
  ESector12Remaining : Outport  Port=231  VectorParamsAs1DForOutWhenUnconnected=off
  NSector1Remaining : Outport  Port=232  VectorParamsAs1DForOutWhenUnconnected=off
  NSector2Remaining : Outport  Port=233  VectorParamsAs1DForOutWhenUnconnected=off
  NSector3Remaining : Outport  Port=234  VectorParamsAs1DForOutWhenUnconnected=off
  NSector4Remaining : Outport  Port=235  VectorParamsAs1DForOutWhenUnconnected=off
  NSector5Remaining : Outport  Port=236  VectorParamsAs1DForOutWhenUnconnected=off
  NSector6Remaining : Outport  Port=237  VectorParamsAs1DForOutWhenUnconnected=off
  NSector7Remaining : Outport  Port=238  VectorParamsAs1DForOutWhenUnconnected=off
  NSector8Remaining : Outport  Port=239  VectorParamsAs1DForOutWhenUnconnected=off
  ESector8Remaining : Outport  Port=240  VectorParamsAs1DForOutWhenUnconnected=off
  NThrottleMapEM : Outport  Port=241  VectorParamsAs1DForOutWhenUnconnected=off
  NThrottleMapOW : Outport  Port=242  VectorParamsAs1DForOutWhenUnconnected=off
  rTorqueSplit : Outport  Port=243  VectorParamsAs1DForOutWhenUnconnected=off
  rTorqueSplitOW : Outport  Port=244  VectorParamsAs1DForOutWhenUnconnected=off
  PRegenMaxEM : Outport  Port=245  VectorParamsAs1DForOutWhenUnconnected=off
  PRegenMaxOW : Outport  Port=246  VectorParamsAs1DForOutWhenUnconnected=off
  rTVMultiplierEM : Outport  Port=247  VectorParamsAs1DForOutWhenUnconnected=off
  rTVMultiplierOW : Outport  Port=248  VectorParamsAs1DForOutWhenUnconnected=off
  rEngineBrakingSplitEM : Outport  Port=249  VectorParamsAs1DForOutWhenUnconnected=off
  rEngineBrakingSplitOW : Outport  Port=250  VectorParamsAs1DForOutWhenUnconnected=off
  PDischargeMaxEM : Outport  Port=251  VectorParamsAs1DForOutWhenUnconnected=off
  PDischargeMaxOW : Outport  Port=252  VectorParamsAs1DForOutWhenUnconnected=off
  PEngineBrakingEM : Outport  Port=253  VectorParamsAs1DForOutWhenUnconnected=off
  PEngineBrakingOW : Outport  Port=254  VectorParamsAs1DForOutWhenUnconnected=off
  NTCKdSelector : Outport  Port=255  VectorParamsAs1DForOutWhenUnconnected=off
  NPCKpSelector : Outport  Port=256  VectorParamsAs1DForOutWhenUnconnected=off
  rTorqueSplitEM : Outport  Port=257  VectorParamsAs1DForOutWhenUnconnected=off
  BTVOnEM : Outport  Port=258  VectorParamsAs1DForOutWhenUnconnected=off
  BTVOnOW : Outport  Port=259  VectorParamsAs1DForOutWhenUnconnected=off
  BDrivetrainCoolingOnEM : Outport  Port=260  VectorParamsAs1DForOutWhenUnconnected=off
  BDrivetrainCoolingOnOW : Outport  Port=261  VectorParamsAs1DForOutWhenUnconnected=off
  BTCOnEM : Outport  Port=262  VectorParamsAs1DForOutWhenUnconnected=off
  BTCOnOW : Outport  Port=263  VectorParamsAs1DForOutWhenUnconnected=off
  BEMSOnEM : Outport  Port=264  VectorParamsAs1DForOutWhenUnconnected=off
  BEMSOnOW : Outport  Port=265  VectorParamsAs1DForOutWhenUnconnected=off
  BSpinningModeOnEM : Outport  Port=266  VectorParamsAs1DForOutWhenUnconnected=off
  BSpinningModeOnOW : Outport  Port=267  VectorParamsAs1DForOutWhenUnconnected=off
  NEventMode : Outport  Port=268  VectorParamsAs1DForOutWhenUnconnected=off
  BInvErrorResetRLCAN3 : Outport  Port=269  VectorParamsAs1DForOutWhenUnconnected=off
  BInvErrorResetFLCAN3 : Outport  Port=270  VectorParamsAs1DForOutWhenUnconnected=off
  BInvErrorResetFRCAN3 : Outport  Port=271  VectorParamsAs1DForOutWhenUnconnected=off
  BInvErrorResetRRCAN3 : Outport  Port=272  VectorParamsAs1DForOutWhenUnconnected=off
  BQuitInvOnFLCAN3 : Outport  Port=273  VectorParamsAs1DForOutWhenUnconnected=off
  BQuitInvOnFRCAN3 : Outport  Port=274  VectorParamsAs1DForOutWhenUnconnected=off
  BQuitInvOnRRCAN3 : Outport  Port=275  VectorParamsAs1DForOutWhenUnconnected=off
  BQuitInvOnRLCAN3 : Outport  Port=276  VectorParamsAs1DForOutWhenUnconnected=off
  BInvDCOnRLOut : Outport  Port=277  VectorParamsAs1DForOutWhenUnconnected=off
  BInvEnableRL : Outport  Port=278  VectorParamsAs1DForOutWhenUnconnected=off
  BInvErrorResetRL : Outport  Port=279  VectorParamsAs1DForOutWhenUnconnected=off
  BInvOnRLOut : Outport  Port=280  VectorParamsAs1DForOutWhenUnconnected=off
  MTorqueLimitNegativeRL : Outport  Port=281  VectorParamsAs1DForOutWhenUnconnected=off
  MTorqueLimitPositiveRL : Outport  Port=282  VectorParamsAs1DForOutWhenUnconnected=off
  MInvRLFinal : Outport  Port=283  VectorParamsAs1DForOutWhenUnconnected=off
  BInvDCOnFLOut : Outport  Port=284  VectorParamsAs1DForOutWhenUnconnected=off
  BInvEnableFL : Outport  Port=285  VectorParamsAs1DForOutWhenUnconnected=off
  BInvErrorResetFL : Outport  Port=286  VectorParamsAs1DForOutWhenUnconnected=off
  BInvOnFLOut : Outport  Port=287  VectorParamsAs1DForOutWhenUnconnected=off
  MTorqueLimitNegativeFL : Outport  Port=288  VectorParamsAs1DForOutWhenUnconnected=off
  MTorqueLimitPositiveFL : Outport  Port=289  VectorParamsAs1DForOutWhenUnconnected=off
  MInvFLFinal : Outport  Port=290  VectorParamsAs1DForOutWhenUnconnected=off
  BInvDCOnRROut : Outport  Port=291  VectorParamsAs1DForOutWhenUnconnected=off
  BInvEnableRR : Outport  Port=292  VectorParamsAs1DForOutWhenUnconnected=off
  BInvErrorResetRR : Outport  Port=293  VectorParamsAs1DForOutWhenUnconnected=off
  BInvOnRROut : Outport  Port=294  VectorParamsAs1DForOutWhenUnconnected=off
  MTorqueLimitNegativeRR : Outport  Port=295  VectorParamsAs1DForOutWhenUnconnected=off
  MTorqueLimitPositiveRR : Outport  Port=296  VectorParamsAs1DForOutWhenUnconnected=off
  MInvRRFinal : Outport  Port=297  VectorParamsAs1DForOutWhenUnconnected=off
  BInvDCOnFROut : Outport  Port=298  VectorParamsAs1DForOutWhenUnconnected=off
  BInvEnableFR : Outport  Port=299  VectorParamsAs1DForOutWhenUnconnected=off
  BInvErrorResetFR : Outport  Port=300  VectorParamsAs1DForOutWhenUnconnected=off
  BInvOnFROut : Outport  Port=301  VectorParamsAs1DForOutWhenUnconnected=off
  MTorqueLimitNegativeFR : Outport  Port=302  VectorParamsAs1DForOutWhenUnconnected=off
  MTorqueLimitPositiveFR : Outport  Port=303  VectorParamsAs1DForOutWhenUnconnected=off
  MInvFRFinal : Outport  Port=304  VectorParamsAs1DForOutWhenUnconnected=off
  wires:
  CAN Rx/21(NPageSelectRotary) -> Bus Creator4/5  "NPageSelectRotary"
  Constant3/1 -> CAN Tx20/11(MRRFinal), CAN Tx20/10(PActual), CAN Tx20/9(MFRFinal), CAN Tx20/8(MRLFinal), CAN Tx20/7(IVTSOut), CAN Tx20/6(MFLFinal), CAN Tx20/5(BOverpower)
  CAN Rx/6(VDamperPotentiometerFR) -> Bus Creator2/7  "VDamperPotentiometerFR"
  CAN Rx/22(NParameterRotary) -> Bus Creator4/6  "NParameterRotary"
  Constant2/1 -> Bus Creator2/1
  CAN Rx/18(BSteeringWheelButton2) -> Bus Creator4/2  "BSteeringWheelButton2"
  Bus Creator3/1 -> Goto8/1
  CAN Rx/9(gVerticalIMU) -> Bus Creator3/2  "gVerticalIMU"
  CAN Rx/4(VBrakeF) -> Bus Creator2/5  "VBrakeF"
  Bus Creator4/1 -> Goto9/1
  CAN Rx/14(gSlipIMU) -> Terminator2/1
  CAN Rx/10(vLongitudinalIMU) -> Bus Creator3/3  "vLongitudinalIMU"
  CAN Rx/12(gLongitudingalIMU) -> Bus Creator3/5
  CAN Rx/13(nYawRateIMU) -> Bus Creator3/6  "nYawRateIMU"
  CAN Rx/7(VDamperPotentiometerFL) -> Bus Creator2/8  "VDamperPotentiometerFL"
  CAN Rx/20(BSteeringWheelButton4) -> Bus Creator4/4  "BSteeringWheelButton4"
  CAN Rx/11(gLateralIMU) -> Bus Creator3/4  "gLateralIMU"
  CAN Rx/17(BSteeringWheelButton1) -> Digital Port Write1/1, Bus Creator4/1  "BSteeringWheelButton1"
  CAN Rx/8(vLateralIMU) -> Bus Creator3/1  "vLateralIMU"
  CAN Rx/16(nRollIMU) -> Terminator/1
  CAN Rx/25(VRegenPaddle2) -> Bus Creator4/9  "VRegenPaddle2"
  CAN Rx/23(NEventModeRotary) -> Bus Creator4/7  "NEventModeRotary"
  Digital Port Read1/1 -> NOT4/1
  CAN Rx/19(BSteeringWheelButton3) -> Bus Creator4/3  "BSteeringWheelButton3"
  Bus Creator2/1 -> Goto6/1
  CAN Rx/15(nPitchIMU) -> Terminator1/1
  CAN Rx/2(VThrottlePedal1) -> Bus Creator2/3  "VThrottlePedal1"
  [MCPInitialized] -> CAN Tx20/1(MCPInitialized)
  NOT4/1 -> Digital Port Write/1, CAN Rx/Enable
  CAN Rx/1(VSteeringAngle) -> Bus Creator2/2  "VSteeringAngle"
  CAN Rx/5(VBrakeR) -> Bus Creator2/6  "VBrakeR"
  CAN Rx/3(VThrottlePedal2) -> Bus Creator2/4  "VThrottlePedal2"
  CAN Rx/24(VRegenPaddle1) -> Bus Creator4/8  "VRegenPaddle1"
  Unit Delay/1 -> NOT/1
  Counter Limited/1 -> Compare To Constant/1
  NOT/1 -> Unit Delay/1
  Subsystem/1(MCPInitialized) -> Goto21/1
  From1/1 -> CAN1_2Bus/1  "InverterFL"
  From/1 -> Model/3
  From4/1 -> CAN1_2Bus/3  "InverterRL"
  From2/1 -> CAN1_2Bus/2  "InverterFR"
  Model/1 -> Goto17/1
  From7/1 -> Bus Creator/3  "IMU"
  From6/1 -> Bus Creator/1  "STW"
  From5/1 -> Bus Creator/2  "DDU7"
  Bus Creator/1 -> Model/2
  From3/1 -> CAN1_2Bus/4  "InverterRR"
  CAN1_2Bus/1 -> Model/1
  0x221/1 -> Bus Selector30/1
  Bus Selector24/2 -> nYawRateErrorActual/1  "<nYawRateErrorActual>"
  Bus Selector13/2 -> BInverterErrorRear/1  "<BInverterErrorRear>"
  Bus Selector9/7 -> MRegenLimited/1  "<MRegenLimited>"
  0x253/1 -> Bus Selector47/1
  Bus Selector6/3 -> aSlipAngleFL/1  "<aSlipAngleFL>"
  Bus Selector13/1 -> NInvState/1  "<NInvState>"
  Bus Selector14/3 -> PInvTemperatureDerateFR/1  "<PInvTemperatureDerateFR>"
  Bus Selector7/3 -> NInvDTCFLOut/1  "<NInvDTCFL>"
  Bus Selector18/7 -> rGrip/1  "<rGrip>"
  Bus Selector7/1 -> NInvDTCRLOut/1  "<NInvDTCRL>"
  Bus Selector2/14 -> BInvErrorResetFRCAN3/1  "<BInvErrorResetFR>"
  Bus Selector2/13 -> BInvErrorResetFLCAN3/1  "<BInvErrorResetFL>"
  Bus Selector8/6 -> BxDamperFROk/1  "<BxDamperFROk>"
  0x300/1 -> Bus Selector33/1
  Bus Selector49/1 -> NBMSState/1  "<NBMSState>"
  Bus Selector1/2 -> PEnergyMeter/1  "<PEnergyMeter>"
  Bus Selector6/4 -> aSlipAngleFR/1  "<aSlipAngleFR>"
  Bus Selector35/1 -> ERemaining/1  "<ERemaining>"
  Bus Selector55/3 -> PRegenMaxEM/1  "<PRegenMaxEM>"
  Bus Selector19/5 -> NABSMultiplierFL/1  "<NABSMultiplierFL>"
  Bus Selector15/6 -> rSlipRatioRLActual/1  "<rSlipRatioRLActual>"
  Bus Selector13/3 -> BInverterErrorFront/1  "<BInverterErrorFront>"
  Bus Selector29/6 -> VCellMinOut/1  "<VCellMin>"
  Bus Selector2/6 -> BPageUp/1  "<BPageUp>"
  0x301/1 -> Bus Selector49/1
  0x702/1 -> Bus Selector53/1
  Bus Selector38/1 -> NSectorGlobal/1  "<NSectorGlobal>"
  Bus Selector4/3 -> MPCDischargeRequested/1  "<MPCDischargeRequested>"
  Bus Selector18/3 -> PDischargeMaxOW/1  "<PDischargeMaxOW>"
  Bus Selector13/8 -> EBudget/1  "<EBudget>"
  Bus Selector2/9 -> BQuitInvOnRRCAN3/1  "<BQuitInvOnRR>"
  0x701/1 -> Bus Selector54/1
  Bus Selector29/3 -> pBrakeR/1  "<pBrakeR>"
  Bus Selector53/6 -> NSector2Remaining/1  "<NSector2Remaining>"
  Bus Selector24/6 -> MTractionControlFLTotal/1  "<MTractionControlFLTotal>"
  Bus Selector6/1 -> FTyreVerticalRL/1  "<FTyreVerticalRL>"
  Bus Selector11/16 -> BBalancingOnOut/1  "<BBalancingOn>"
  Bus Selector55/2 -> PRegenMax/1  "<PRegenMax>"
  Bus Selector30/5 -> PDischargeDerate/1  "<PDischargeDerate>"
  Bus Selector31/3 -> BReadyToDriveBuzzer/1  "<BReadyToDriveBuzzer>"
  Bus Selector14/6 -> IBMSHallEffectOut/1  "<IBMSHallEffect>"
  0x212/1 -> Bus Selector9/1
  Bus Selector13/9 -> BTVOK/1  "<BTVOK>"
  Bus Selector2/1 -> vWheelFL/1  "<vWheelFL>"
  Bus Selector33/3 -> TMotorRLOut/1  "<TMotorRL>"
  Bus Selector31/1 -> BPCComplete/1  "<BPCComplete>"
  Bus Selector30/8 -> PDischargeLimit/1  "<PDischargeLimit>"
  Bus Selector12/4 -> MDriverDischargeRequested/1  "<MDriverDischargeRequested>"
  0x210/1 -> Bus Selector5/1
  Bus Selector10/5 -> aCamberRL/1  "<aCamberRL>"
  Bus Selector4/2 -> PPCProportionalTermDischarge/1  "<PPCProportionalTermDischarge>"
  0x703/1 -> Bus Selector38/1
  Bus Selector/7 -> BBrakeError/1  "<BBrakeError>"
  Bus Selector13/10 -> sSector/1  "<sSector>"
  Bus Selector11/15 -> rSOE/1  "<rSOE>"
  Bus Selector/5 -> IIVTSOut/1  "<IIVTS>"
  Bus Selector30/4 -> BSpeedDerateOn/1  "<BSpeedDerateOn>"
  Bus Selector38/3 -> NSector3Remaining/1  "<NSector3Remaining>"
  Bus Selector6/6 -> aSlipAngleRR/1  "<aSlipAngleRR>"
  Bus Selector10/3 -> aCamberFL/1  "<aCamberFL>"
  Bus Selector34/5 -> ESector4Remaining/1  "<ESector4Remaining>"
  Bus Selector19/3 -> NTractionControlMultiplierRL/1  "<NTractionControlMultiplierRL>"
  Bus Selector53/3 -> ESector11Remaining/1  "<ESector11Remaining>"
  Bus Selector8/13 -> PPCRegenRequested/1  "<PPCRegenRequested>"
  Bus Selector19/2 -> MTorqueDistributionRR/1  "<MTorqueDistributionRR>"
  Bus Selector13/5 -> TInvRLOut/1  "<TInvRL>"
  0x202/1 -> Bus Selector/1
  Bus Selector47/3 -> PTSTemperatureDerateFL/1  "<PTSTemperatureDerateFL>"
  Bus Selector11/23 -> NLap/1  "<NLap>"
  Bus Selector11/5 -> BDrivetrainCoolingOnOW/1  "<BDrivetrainCoolingOnOW>"
  Bus Selector14/1 -> sChassis/1  "<sChassis>"
  Bus Selector3/5 -> rThrottlePedal/1  "<rThrottlePedal>"
  Bus Selector18/5 -> PEngineBrakingEM/1  "<PEngineBrakingEM>"
  Bus Selector49/6 -> TCellMinOut/1  "<TCellMin>"
  Bus Selector18/2 -> PDischargeMaxEM/1  "<PDischargeMaxEM>"
  Bus Selector30/7 -> PRegenRequested/1  "<PRegenRequested>"
  Bus Selector/2 -> MFRFinal/1  "<MFRFinal>"
  0x211/1 -> Bus Selector12/1
  Bus Selector42/2 -> PMotorTemperatureDerate/1  "<PMotorTemperatureDerate>"
  Bus Selector53/4 -> ESector12Remaining/1  "<ESector12Remaining>"
  Bus Selector55/10 -> rEngineBrakingSplitOW/1  "<rEngineBrakingSplitOW>"
  Bus Selector/9 -> BOverpower/1  "<BOverpower>"
  Bus Selector8/10 -> BCalibrationOn/1  "<BCalibrationOn>"
  Bus Selector8/5 -> BxDamperFLOk/1  "<BxDamperFLOk>"
  Bus Selector4/1 -> tPedalOverlap/1  "<tPedalOverlap>"
  Bus Selector15/7 -> FTyreVerticalFR/1  "<FTyreVerticalFR>"
  Bus Selector11/3 -> BDrivetrainCoolingOn/1  "<BDrivetrainCoolingOn>"
  Bus Selector/1 -> MFLFinal/1  "<MFLFinal>"
  Bus Selector19/1 -> tThrottleError/1  "<tThrottleError>"
  Bus Selector49/2 -> TInvRROut/1  "<TInvRR>"
  Bus Selector18/4 -> PEngineBraking/1  "<PEngineBraking>"
  Bus Selector8/3 -> BAppsOK/1  "<BAppsOK>"
  Bus Selector9/2 -> MTorqueVectoringFR/1  "<MTorqueVectoringFR>"
  Bus Selector55/1 -> rTorqueSplitOW/1  "<rTorqueSplitOW>"
  Bus Selector/3 -> MRLFinal/1  "<MRLFinal>"
  Bus Selector14/2 -> PInvTemperatureDerate/1  "<PInvTemperatureDerate>"
  Bus Selector30/9 -> PRegenLimit/1  "<PRegenLimit>"
  Bus Selector11/27 -> NThrottleMapEM/1  "<NThrottleMapEM>"
  Bus Selector55/12 -> BReadyToDrive/1  "<BReadyToDrive>"
  Bus Selector14/5 -> PInvTemperatureDerateRR/1  "<PInvTemperatureDerateRR>"
  Bus Selector55/7 -> rTVMultiplierOW/1  "<rTVMultiplierOW>"
  Bus Selector11/1 -> BTVOnEM/1  "<BTVOnEM>"
  Bus Selector12/6 -> PPCIntegralTermDischarge/1  "<PPCIntegralTermDischarge>"
  Bus Selector8/9 -> BIMUError/1  "<BIMUError>"
  Bus Selector2/5 -> rThrottlePedal1/1  "<rThrottlePedal1>"
  Bus Selector11/24 -> NEventMode/1  "<NEventMode>"
  Bus Selector11/21 -> BBMSP0AC0Out/1  "<BBMSP0AC0>"
  Bus Selector54/6 -> ESector6Remaining/1  "<ESector6Remaining>"
  Bus Selector18/11 -> MRegenMax/1  "<MRegenMax>"
  0x254/1 -> Bus Selector48/1
  Bus Selector8/2 -> BPedalOverlap/1  "<BPedalOverlap>"
  Bus Selector8/4 -> BRegenOn/1  "<BRegenOn>"
  0x1A2/1 -> Bus Selector18/1
  Bus Selector12/3 -> PHighCellVoltageRegenDerate/1  "<PHighCellVoltageRegenDerate>"
  Bus Selector29/2 -> pBrakeF/1  "<pBrakeF>"
  Bus Selector2/11 -> BInvErrorResetRLCAN3/1  "<BInvErrorResetRL>"
  Bus Selector9/1 -> MTorqueVectoringFL/1  "<MTorqueVectoringFL>"
  Bus Selector19/4 -> NTractionControlMultiplierRR/1  "<NTractionControlMultiplierRR>"
  Bus Selector35/7 -> aRollAngle/1  "<aRollAngle>"
  Bus Selector35/3 -> aCamberGainRollF/1  "<aCamberGainRollF>"
  Bus Selector3/6 -> BPageDown/1  "<BPageDown>"
  0x700/1 -> Bus Selector34/1
  Bus Selector29/7 -> PSOCDischargeDerate/1  "<PSOCDischargeDerate>"
  Bus Selector33/4 -> VDCInvRLOut/1  "<VDCInvRL>"
  Bus Selector2/7 -> BQuitInvOnRLCAN3/1  "<BQuitInvOnRL>"
  0x250/1 -> Bus Selector14/1
  Bus Selector53/2 -> ESector10Remaining/1  "<ESector10Remaining>"
  Bus Selector8/15 -> BEMSDriverSignal1/1  "<BEMSDriverSignal1>"
  Bus Selector38/6 -> NSector6Remaining/1  "<NSector6Remaining>"
  0x1A0/1 -> Bus Selector11/1
  Bus Selector4/7 -> NTractionControlMultiplierFL/1  "<NTractionControlMultiplierFL>"
  Bus Selector7/4 -> NInvDTCFROut/1  "<NInvDTCFR>"
  Bus Selector31/7 -> BInvLVOn/1  "<BInvLVOn>"
  Bus Selector12/1 -> aSteeringAngle/1  "<aSteeringAngle>"
  Bus Selector35/6 -> aCamberGainHeaveR/1  "<aCamberGainHeaveR>"
  0x217/1 -> Bus Selector6/1
  Bus Selector18/1 -> PDischargeMax/1  "<PDischargeMax>"
  0x214/1 -> Bus Selector19/1
  Bus Selector55/5 -> rTVMultiplier/1  "<rTVMultiplier>"
  Bus Selector48/3 -> xHeaveTravelR/1  "<xHeaveTravelR>"
  Bus Selector5/1 -> pBrakeMax/1  "<pBrakeMax>"
  Bus Selector29/1 -> NCarState/1  "<NCarState>"
  Bus Selector33/2 -> TInvMax/1  "<TInvMax>"
  Bus Selector38/8 -> NSector8Remaining/1  "<NSector8Remaining>"
  Bus Selector31/2 -> BBrakeLight/1  "<BBrakeLight>"
  Bus Selector2/4 -> nMotorFROut/1  "<nMotorFR>"
  Bus Selector34/2 -> ESector1Remaining/1  "<ESector1Remaining>"
  Bus Selector6/5 -> aSlipAngleRL/1  "<aSlipAngleRL>"
  Bus Selector4/5 -> MPCRegenRequested/1  "<MPCRegenRequested>"
  Bus Selector9/6 -> MTorqueDistributionFR/1  "<MTorqueDistributionFR>"
  Bus Selector33/1 -> TMotorMax/1  "<TMotorMax>"
  Bus Selector11/8 -> BTCOnOW/1  "<BTCOnOW>"
  Bus Selector1/1 -> vChassis/1  "<vChassis>"
  Bus Selector15/2 -> MTractionControlRRTotal/1  "<MTractionControlRRTotal>"
  Bus Selector5/2 -> rRegenPaddle/1  "<rRegenPaddle>"
  Bus Selector8/7 -> BxDamperRLOk/1  "<BxDamperRLOk>"
  0x302/1 -> Bus Selector13/1
  Bus Selector11/4 -> BDrivetrainCoolingOnEM/1  "<BDrivetrainCoolingOnEM>"
  0x205/1 -> Bus Selector2/1
  0x206/1 -> Bus Selector3/1
  Bus Selector10/2 -> rSlipRatioOptimal/1  "<rSlipRatioOptimal>"
  Bus Selector5/3 -> xDamperFL/1  "<xDamperFL>"
  Bus Selector18/6 -> PEngineBrakingOW/1  "<PEngineBrakingOW>"
  Bus Selector48/1 -> ESector/1  "<ESector>"
  Bus Selector54/5 -> ESector5Remaining/1  "<ESector5Remaining>"
  Bus Selector2/12 -> BInvErrorResetRRCAN3/1  "<BInvErrorResetRR>"
  Bus Selector30/10 -> PPCDischargeRequested/1  "<PPCDischargeRequested>"
  Bus Selector19/6 -> NABSMultiplierFR/1  "<NABSMultiplierFR>"
  Bus Selector42/3 -> PMotorTemperatureDerateFR/1  "<PMotorTemperatureDerateFR>"
  Bus Selector11/28 -> NThrottleMapOW/1  "<NThrottleMapOW>"
  0x1A1/1 -> Bus Selector55/1
  Bus Selector18/10 -> NPCKpSelector/1  "<NPCKpSelector>"
  Bus Selector19/8 -> FTyreVerticalFL/1  "<FTyreVerticalFL>"
  Bus Selector13/7 -> VDCAccumulatorOut/1  "<VDCAccumulator>"
  Bus Selector24/5 -> MTractionControlFRTotal/1  "<MTractionControlFRTotal>"
  Bus Selector30/2 -> rSpeedRegenDerateFR/1  "<rSpeedRegenDerateFR>"
  Bus Selector35/2 -> FTotalDownforce/1  "<FTotalDownforce>"
  0x207/1 -> Bus Selector7/1
  Bus Selector8/16 -> BEMSDriverSignal2/1  "<BEMSDriverSignal2>"
  Bus Selector31/5 -> BMotorRBHFanOn/1  "<BMotorRBHFanOn>"
  Bus Selector9/3 -> MTorqueVectoringRL/1  "<MTorqueVectoringRL>"
  Bus Selector11/14 -> BSpinningModeOnOW/1  "<BSpinningModeOnOW>"
  Bus Selector/10 -> BDischargeAllowed/1  "<BDischargeAllowed>"
  Bus Selector11/19 -> BBMSP0A10Out/1  "<BBMSP0A10>"
  Bus Selector10/1 -> MTotalRequested/1  "<MTotalRequested>"
  Bus Selector3/4 -> nMotorRROut/1  "<nMotorRR>"
  0x603/1 -> Bus Selector31/1
  Bus Selector2/8 -> BQuitInvOnFLCAN3/1  "<BQuitInvOnFL>"
  Bus Selector11/10 -> BEMSOnEM/1  "<BEMSOnEM>"
  Bus Selector29/4 -> tAppsTimer/1  "<tAppsTimer>"
  Bus Selector5/9 -> BDataMark/1  "<BDataMark>"
  Bus Selector15/4 -> rSlipRatioFLActual/1  "<rSlipRatioFLActual>"
  Bus Selector33/5 -> TMotorRROut/1  "<TMotorRR>"
  Bus Selector12/5 -> MDriverRegenRequested/1  "<MDriverRegenRequested>"
  Bus Selector11/2 -> BTVOnOW/1  "<BTVOnOW>"
  0x203/1 -> Bus Selector1/1
  Bus Selector10/6 -> aCamberRR/1  "<aCamberRR>"
  Bus Selector34/3 -> ESector2Remaining/1  "<ESector2Remaining>"
  Bus Selector48/2 -> xHeaveTravelF/1  "<xHeaveTravelF>"
  Bus Selector4/6 -> MDischargeLimited/1  "<MDischargeLimited>"
  Bus Selector30/3 -> rSpeedRegenDerateFL/1  "<rSpeedRegenDerateFL>"
  Bus Selector13/4 -> BErrorReset/1  "<BErrorReset>"
  0x213/1 -> Bus Selector4/1
  Bus Selector11/7 -> BTCOnEM/1  "<BTCOnEM>"
  Bus Selector12/2 -> PLowCellVoltageDischargeDerate/1  "<PLowCellVoltageDischargeDerate>"
  Bus Selector11/22 -> BBMSP0AFAOut/1  "<BBMSP0AFA>"
  Bus Selector24/4 -> MTractionControlRLTotal/1  "<MTractionControlRLTotal>"
  Bus Selector/8 -> BThrottleError/1  "<BThrottleError>"
  Bus Selector11/6 -> BTCOn/1  "<BTCOn>"
  Bus Selector47/2 -> PTSTemperatureDerateFR/1  "<PTSTemperatureDerateFR>"
  Bus Selector49/5 -> TCellMaxOut/1  "<TCellMax>"
  Bus Selector5/8 -> tIMUError/1  "<tIMUError>"
  0x223/1 -> Bus Selector8/1
  Bus Selector38/7 -> NSector7Remaining/1  "<NSector7Remaining>"
  Bus Selector3/3 -> nMotorRLOut/1  "<nMotorRL>"
  Bus Selector15/5 -> rSlipRatioFRActual/1  "<rSlipRatioFRActual>"
  Bus Selector13/6 -> TMotorFROut/1  "<TMotorFR>"
  Bus Selector11/18 -> BBMSP0A0EOut/1  "<BBMSP0A0E>"
  Bus Selector38/5 -> NSector5Remaining/1  "<NSector5Remaining>"
  Bus Selector38/4 -> NSector4Remaining/1  "<NSector4Remaining>"
  Bus Selector8/11 -> PSOCRegenDerate/1  "<PSOCRegenDerate>"
  Bus Selector2/10 -> BQuitInvOnFRCAN3/1  "<BQuitInvOnFR>"
  Bus Selector47/1 -> PMotorTemperatureDerateRL/1  "<PMotorTemperatureDerateRL>"
  Bus Selector8/17 -> BEMSDriverSignal3/1  "<BEMSDriverSignal3>"
  Bus Selector9/5 -> MTorqueDistributionFL/1  "<MTorqueDistributionFL>"
  Bus Selector35/5 -> aCamberGainHeaveF/1  "<aCamberGainHeaveF>"
  Bus Selector2/3 -> nMotorFLOut/1  "<nMotorFL>"
  Bus Selector31/6 -> BInverterFanOn/1  "<BInverterFanOn>"
  Bus Selector9/4 -> MTorqueVectoringRR/1  "<MTorqueVectoringRR>"
  Bus Selector55/4 -> PRegenMaxOW/1  "<PRegenMaxOW>"
  Bus Selector47/6 -> PHighCellTemperatureDerate/1  "<PHighCellTemperatureDerate>"
  Bus Selector38/9 -> ESector8Remaining/1  "<ESector8Remaining>"
  Bus Selector14/4 -> PInvTemperatureDerateFL/1  "<PInvTemperatureDerateFL>"
  Bus Selector55/13 -> BTVOn/1  "<BTVOn>"
  Bus Selector15/1 -> NABSMultiplierRR/1  "<NABSMultiplierRR>"
  Bus Selector49/4 -> TInvFROut/1  "<TInvFR>"
  Bus Selector30/1 -> rSpeedRegenDerateRL/1  "<rSpeedRegenDerateRL>"
  Bus Selector11/25 -> rTorqueSplit/1  "<rTorqueSplit>"
  Bus Selector5/5 -> xDamperRL/1  "<xDamperRL>"
  Bus Selector54/7 -> ESector7Remaining/1  "<ESector7Remaining>"
  Bus Selector55/6 -> rTVMultiplierEM/1  "<rTVMultiplierEM>"
  Bus Selector8/18 -> FLongitudinalLoadTransfer/1  "<FLongitudinalLoadTransfer>"
  Bus Selector53/1 -> ESector9Remaining/1  "<ESector9Remaining>"
  Bus Selector42/5 -> PMotorTemperatureDerateRR/1  "<PMotorTemperatureDerateRR>"
  Bus Selector54/1 -> NSector9Remaining/1  "<NSector9Remaining>"
  Bus Selector11/13 -> BSpinningModeOnEM/1  "<BSpinningModeOnEM>"
  Bus Selector2/2 -> vWheelFR/1  "<vWheelFR>"
  Bus Selector38/2 -> NSectorLap/1  "<NSectorLap>"
  Bus Selector31/4 -> BAccuFanOn/1  "<BAccuFanOn>"
  Bus Selector10/4 -> aCamberFR/1  "<aCamberFR>"
  Bus Selector4/8 -> NTractionControlMultiplierFR/1  "<NTractionControlMultiplierFR>"
  Bus Selector42/1 -> PInvTemperatureDerateRL/1  "<PInvTemperatureDerateRL>"
  Bus Selector4/4 -> PPCProportionalTermRegen/1  "<PPCProportionalTermRegen>"
  Bus Selector15/3 -> MTotalFinal/1  "<MTotalFinal>"
  Bus Selector11/20 -> BBMSP0A80Out/1  "<BBMSP0A80>"
  0x222/1 -> Bus Selector10/1
  Bus Selector54/2 -> NSector10Remaining/1  "<NSector10Remaining>"
  Bus Selector55/9 -> rEngineBrakingSplitEM/1  "<rEngineBrakingSplitEM>"
  Bus Selector12/7 -> PPCIntegralTermRegen/1  "<PPCIntegralTermRegen>"
  Bus Selector35/4 -> aCamberGainRollR/1  "<aCamberGainRollR>"
  Bus Selector34/4 -> ESector3Remaining/1  "<ESector3Remaining>"
  Bus Selector42/7 -> aCamberGainSteerFR/1  "<aCamberGainSteerFR>"
  0x220/1 -> Bus Selector29/1
  Bus Selector8/12 -> rSpeedRegenDerateRR/1  "<rSpeedRegenDerateRR>"
  Bus Selector11/12 -> BSpinningModeOn/1  "<BSpinningModeOn>"
  Bus Selector24/7 -> rSlipRatioRRActual/1  "<rSlipRatioRRActual>"
  Bus Selector10/7 -> FTotalLateralLoadTransfer/1  "<FTotalLateralLoadTransfer>"
  Bus Selector11/17 -> BBMSP0A0COut/1  "<BBMSP0A0C>"
  Bus Selector8/1 -> BBrakeOn/1  "<BBrakeOn>"
  Bus Selector54/4 -> NSector12Remaining/1  "<NSector12Remaining>"
  Bus Selector7/2 -> NInvDTCRROut/1  "<NInvDTCRR>"
  Bus Selector5/4 -> xDamperFR/1  "<xDamperFR>"
  Bus Selector34/1 -> ETotalRequested/1  "<ETotalRequested>"
  Bus Selector11/9 -> BEMSOn/1  "<BEMSOn>"
  0x216/1 -> Bus Selector15/1
  Bus Selector55/8 -> rEngineBrakingSplit/1  "<rEngineBrakingSplit>"
  Bus Selector47/5 -> PTSTemperatureDerateRL/1  "<PTSTemperatureDerateRL>"
  Bus Selector49/3 -> TInvFLOut/1  "<TInvFL>"
  Bus Selector5/6 -> xDamperRR/1  "<xDamperRR>"
  Bus Selector49/7 -> rSplitRear/1  "<rSplitRear>"
  Bus Selector18/12 -> rTorqueSplitEM/1  "<rTorqueSplitEM>"
  0x215/1 -> Bus Selector24/1
  Bus Selector47/4 -> PTSTemperatureDerateRR/1  "<PTSTemperatureDerateRR>"
  Bus Selector3/1 -> vWheelRL/1  "<vWheelRL>"
  Bus Selector24/3 -> MTorqueDistributionRL/1  "<MTorqueDistributionRL>"
  Bus Selector18/9 -> NTCKdSelector/1  "<NTCKdSelector>"
  0x251/1 -> Bus Selector42/1
  Bus Selector42/4 -> PMotorTemperatureDerateFL/1  "<PMotorTemperatureDerateFL>"
  Bus Selector54/3 -> NSector11Remaining/1  "<NSector11Remaining>"
  Bus Selector42/6 -> aCamberGainSteerFL/1  "<aCamberGainSteerFL>"
  Bus Selector5/7 -> BIMUOk/1  "<BIMUOK>"
  0x252/1 -> Bus Selector35/1
  Bus Selector11/26 -> NThrottleMap/1  "<NThrottleMap>"
  Bus Selector53/5 -> NSector1Remaining/1  "<NSector1Remaining>"
  Bus Selector8/8 -> BxDamperRROk/1  "<BxDamperRROk>"
  Bus Selector29/5 -> VCellMaxOut/1  "<VCellMax>"
  Bus Selector11/11 -> BEMSOnOW/1  "<BEMSOnOW>"
  Bus Selector33/6 -> TMotorFLOut/1  "<TMotorFL>"
  Bus Selector/6 -> PActual/1  "<PActual>"
  Bus Selector30/6 -> PRegenDerate/1  "<PRegenDerate>"
  Bus Selector18/8 -> EOffset/1  "<EOffset>"
  Bus Selector/4 -> MRRFinal/1  "<MRRFinal>"
  Bus Selector19/7 -> NABSMultiplierRL/1  "<NABSMultiplierRL>"
  Bus Selector6/2 -> FTyreVerticalRR/1  "<FTyreVerticalRR>"
  Bus Selector8/14 -> PDischargeLimited/1  "<PDischargeLimited>"
  Bus Selector24/1 -> tBrakeError/1  "<tBrakeError>"
  Bus Selector3/2 -> vWheelRR/1  "<vWheelRR>"
  Bus Selector55/11 -> rSOC/1  "<rSOC>"
  Bus Selector23/6 -> MTorqueLimitPositiveFR/1  "<MTorqueLimitPositiveFR>"
  INV3_Recieve_1/1 -> Bus Selector22/1
  Bus Selector22/2 -> BInvEnableRR/1  "<BInvEnableRR>"
  Bus Selector22/1 -> BInvDCOnRROut/1  "<BInvDCOnRROut>"
  Bus Selector21/5 -> MTorqueLimitNegativeFL/1  "<MTorqueLimitNegativeFL>"
  Bus Selector21/2 -> BInvEnableFL/1  "<BInvEnableFL>"
  Bus Selector23/5 -> MTorqueLimitNegativeFR/1  "<MTorqueLimitNegativeFR>"
  Bus Selector20/4 -> BInvOnRLOut/1  "<BInvOnRLOut>"
  Bus Selector20/2 -> BInvEnableRL/1  "<BInvEnableRL>"
  INV4_Recieve_1/1 -> Bus Selector23/1
  Bus Selector23/2 -> BInvEnableFR/1  "<BInvEnableFR>"
  Bus Selector21/6 -> MTorqueLimitPositiveFL/1  "<MTorqueLimitPositiveFL>"
  Bus Selector23/1 -> BInvDCOnFROut/1  "<BInvDCOnFROut>"
  Bus Selector23/7 -> MInvFRFinal/1  "<MFRFinal>"
  Bus Selector20/5 -> MTorqueLimitNegativeRL/1  "<MTorqueLimitNegativeRL>"
  Bus Selector20/7 -> MInvRLFinal/1  "<MRLFinal>"
  Bus Selector21/1 -> BInvDCOnFLOut/1  "<BInvDCOnFLOut>"
  INV2_Recieve_1/1 -> Bus Selector21/1
  Bus Selector22/4 -> BInvOnRROut/1  "<BInvOnRROut>"
  Bus Selector21/7 -> MInvFLFinal/1  "<MFLFinal>"
  Bus Selector20/1 -> BInvDCOnRLOut/1  "<BInvDCOnRLOut>"
  Bus Selector20/3 -> BInvErrorResetRL/1  "<BInvErrorResetRL>"
  Bus Selector22/6 -> MTorqueLimitPositiveRR/1  "<MTorqueLimitPositiveRR>"
  Bus Selector23/4 -> BInvOnFROut/1  "<BInvOnFROut>"
  Bus Selector22/3 -> BInvErrorResetRR/1  "<BInvErrorResetRR>"
  Bus Selector22/5 -> MTorqueLimitNegativeRR/1  "<MTorqueLimitNegativeRR>"
  INV1_Recieve_1/1 -> Bus Selector20/1
  Bus Selector20/6 -> MTorqueLimitPositiveRL/1  "<MTorqueLimitPositiveRL>"
  Bus Selector22/7 -> MInvRRFinal/1  "<MRRFinal>"
  Bus Selector23/3 -> BInvErrorResetFR/1  "<BInvErrorResetFR>"
  Bus Selector21/4 -> BInvOnFLOut/1  "<BInvOnFLOut>"
  Bus Selector21/3 -> BInvErrorResetFL/1  "<BInvErrorResetFL>"
  TMotorRR/1 -> Bus Creator19/11  "TMotorRR"
  BQuitInvOnRL/1 -> Bus Creator17/6  "BQuitInvOnRL"
  BInvDCOnFLIn/1 -> Bus Creator14/2  "BInvDCOnFLIn"
  BInvSysReadyFL/1 -> Bus Creator14/7  "BInvSysReadyFL"
  BInvWarnRL/1 -> Bus Creator17/8  "BInvWarnRL"
  MMotorMeasuredRR/1 -> Bus Creator19/9  "MMotorMeasuredRR"
  nMotorFL/1 -> Bus Creator14/1  "nMotorFL"
  BInvQuitDcOnFR/1 -> Bus Creator15/5  "BInvQuitDcOnFR"
  Bus Creator18/1 -> Goto4/1
  NInvDTCRL/1 -> Bus Creator17/10  "NInvDTCRL"
  BInvErrorFR/1 -> Bus Creator15/3  "BInvErrorFR"
  VCellMax/1 -> Bus Creator18/6  "VCellMax"
  BInvWarnRR/1 -> Bus Creator19/8  "BInvWarnRR"
  BBMSP0A0C/1 -> Bus Creator18/12  "BBMSP0A0C"
  Bus Creator17/1 -> Goto/1
  BBMSP0A10/1 -> Bus Creator18/14  "BBMSP0A10"
  BInvQuitDcOnRR/1 -> Bus Creator19/5  "BInvQuitDcOnRR"
  TCellMin/1 -> Bus Creator18/4  "TCellMin"
  BQuitInvOnFR/1 -> Bus Creator15/6  "BQuitInvOnFR"
  BInvErrorRL/1 -> Bus Creator17/3  "BInvErrorRL"
  BInvDCOnRLIn/1 -> Bus Creator17/2  "BInvDCOnRLIn"
  VDCAccumulator/1 -> Bus Creator18/3  "VDCAccumulator"
  BInvWarnFR/1 -> Bus Creator15/8  "BInvWarnFR"
  VDCInvRL/1 -> Bus Creator17/12  "VDCInvRL"
  IBMSDCL/1 -> Bus Creator18/8  "IBMSDCL"
  BInvSysReadyFR/1 -> Bus Creator15/7  "BInvSysReadyFR"
  IIVTS/1 -> Bus Creator18/1  "IIVTS"
  TInvRR/1 -> Bus Creator19/13  "TInvRR"
  VDCInvRR/1 -> Bus Creator19/12  "VDCInvRR"
  BBMSP0AC0/1 -> Bus Creator18/16  "BBMSP0AC0"
  BInvQuitDcOnFL/1 -> Bus Creator14/5  "BInvQuitDcOnFL"
  nMotorFR/1 -> Bus Creator15/1  "nMotorFR"
  BInvSysReadyRL/1 -> Bus Creator17/7  "BInvSysReadyRL"
  VDCInvFL/1 -> Bus Creator14/12  "VDCInvFL"
  BBMSP0A0E/1 -> Bus Creator18/13  "BBMSP0A0E"
  MMotorMeasuredFL/1 -> Bus Creator14/9  "MMotorMeasuredFL"
  Bus Creator14/1 -> Goto2/1
  BInvOnFRIn/1 -> Bus Creator15/4  "BInvOnFRIn"
  BInvOnFLIn/1 -> Bus Creator14/4  "BInvOnFLIn"
  VDCInvFR/1 -> Bus Creator15/12  "VDCInvFR"
  Bus Creator15/1 -> Goto3/1
  BInvOnRLIn/1 -> Bus Creator17/4  "BInvOnRLIn"
  NInvDTCFR/1 -> Bus Creator15/10  "NInvDTCFR"
  BInvErrorRR/1 -> Bus Creator19/3  "BInvErrorRR"
  BQuitInvOnFL/1 -> Bus Creator14/6  "BQuitInvOnFL"
  RCellAverage/1 -> Bus Creator18/10  "RCellAverage"
  BInvWarnFL/1 -> Bus Creator14/8  "BInvWarnFL"
  Bus Creator19/1 -> Goto1/1
  MMotorMeasuredFR/1 -> Bus Creator15/9  "MMotorMeasuredFR"
  MMotorMeasuredRL/1 -> Bus Creator17/9  "MMotorMeasuredRL"
  nMotorRL/1 -> Bus Creator17/1  "nMotorRL"
  BInvQuitDcOnRL/1 -> Bus Creator17/5  "BInvQuitDcOnRL"
  nMotorRR/1 -> Bus Creator19/1  "nMotorRR"
  BBalancingOn/1 -> Bus Creator18/11  "BBalancingOn"
  BBMSP0AFA/1 -> Bus Creator18/17  "BBMSP0AFA"
  TMotorFL/1 -> Bus Creator14/11  "TMotorFL"
  NInvDTCRR/1 -> Bus Creator19/10  "NInvDTCRR"
  TInvRL/1 -> Bus Creator17/13  "TInvRL"
  BInvDCOnFRIn/1 -> Bus Creator15/2  "BInvDCOnFRIn"
  TCellMax/1 -> Bus Creator18/7  "TCellMax"
  VCellMin/1 -> Bus Creator18/9  "VCellMin"
  IBMSHallEffect/1 -> Bus Creator18/2  "IBMSHallEffect"
  NInvDTCFL/1 -> Bus Creator14/10  "NInvDTCFL"
  TInvFR/1 -> Bus Creator15/13  "TInvFR"
  TInvFL/1 -> Bus Creator14/13  "TInvFL"
  TMotorRL/1 -> Bus Creator17/11  "TMotorRL"
  BInvErrorFL/1 -> Bus Creator14/3  "BInvErrorFL"
  TMotorFR/1 -> Bus Creator15/11  "TMotorFR"
  VCellAverage/1 -> Bus Creator18/5  "VCellAverage"
  BInvDCOnRRIn/1 -> Bus Creator19/2  "BInvDCOnRRIn"
  BInvSysReadyRR/1 -> Bus Creator19/7  "BInvSysReadyRR"
  BBMSP0A80/1 -> Bus Creator18/15  "BBMSP0A80"
  BQuitInvOnRR/1 -> Bus Creator19/6  "BQuitInvOnRR"
  BInvOnRRIn/1 -> Bus Creator19/4  "BInvOnRRIn"
  Digital Port Read3/1 -> NOT1/1
  NOT1/1 -> Digital Port Write2/1, CAN Rx1/Enable
  CAN Rx1/5(ID) -> CAN Tx20/12(Number1), Data Type Conversion/1
  CAN Rx1/6(Length) -> ?
  Compare To Constant1/1 -> Digital Port Write3/1
  CAN Rx1/7(Byte) -> CAN Tx20/14(Number3)
  CAN Rx1/8(Byte1) -> CAN Tx20/15(Number4)
  CAN Rx1/4(VADC1) -> CAN Tx20/13(Number2)
  Data Type Conversion/1 -> Compare To Constant1/1
  Subsystem1/1(MCPInitialized) -> [MCPInitialized]
